simulink model "Test2_1"  (R2021a)
(part 1 of 2)
settings: Solver=FixedStepAuto  StartTime=0  StopTime=0.2  FixedStep=0.2  RelTol=1e-3
libraries: spsDistributedParametersLineLib x92, spsThreePhaseSeriesRLCLoadLib x30, spsThreePhaseVIMeasurementLib x4, spsGroundLib x1, spsThreePhaseSourceLib x1, spsSeriesRLCBranchLib x1, spspowerguiLib x1
settings Model: Creator=Admin  LastModifiedBy=Admin

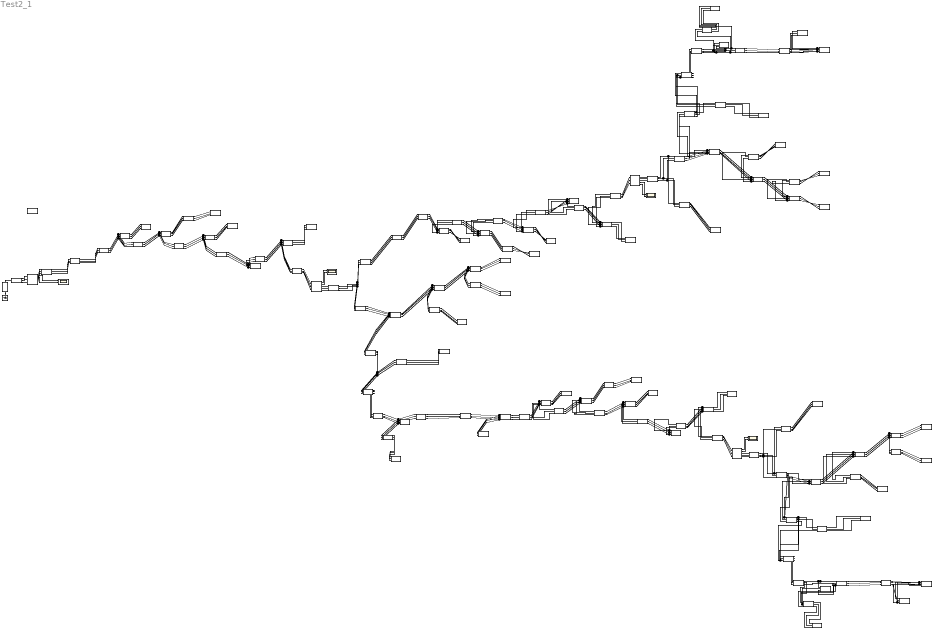
== system Test2_1 ==
  Ground : spsGroundLib/Ground  LConnTagsString=a
  Line 1 : spsDistributedParametersLineLib/Distributed Parameters Line  Phases=3  Length=1.11  Frequency=50  Resistance=[0.502970710632245 0.0486237908083191 0.0486712220507153;0.0486237908083191 0.502875844822084 0.0486237934466192;0.0486712220507153 0.0486237934466192 0.502970710632245]  Inductance=[0.00286900545038753 0.00133270803418135 0.00132951476746136;0.00133270803418135 0.00286931445999602 0.00133799988507366;0.00132951476746136 0.00133799988507366 0.00286900545038753]  Capacitance=[8.11484299003193e-09 -1.94249816214699e-09 -1.86930692621136e-09;-1.94249816214699e-09 8.0425699231653e-09 -1.98049571960044e-09;-1.86930692621136e-09 -1.98049571960044e-09 8.13337738722527e-09]  x1=[183.490948188185 4216.96054972605 4216.80340700784;314.159265358979 314.159265358979 314.159265358979;0.881345582847074 1.88304842426721 -2.82810315151267]  x2=[183.491209806206 4216.96449324722 4216.80735926271;314.159265358979 314.159265358979 314.159265358979;0.881345090635743 1.88304754646511 -2.82810403687592]  x3=[0.160865210922633 10.7270372245128 10.8089995229869;314.159265358979 314.159265358979 314.159265358979;0.879656680482595 1.88168039127429 -2.82947272736112]  x4=[0.160865210931406 10.7270372277551 10.8089995262806;314.159265358979 314.159265358979 314.159265358979;0.881345090559868 1.88304754646581 -2.82810403687496]  x5=5.37516004033389e-06  V1=ones(3,3)  V2=ones(3,3)  I1=ones(3,3)  I2=ones(3,3)  nHarmo=1  Measurements=None  Decoupling=off  VsMag0=0  VrMag0=0  VsAngle0=0  VrAngle0=0  IsMag0=0  IrMag0=0  IsAngle0=0  IrAngle0=0
      settings: SourceProductBaseCode=PS
  Line 10 : spsDistributedParametersLineLib/Distributed Parameters Line  Phases=3  Length=0.02  Frequency=50  Resistance=[0.646656091154803 0.0486237908083191 0.0486712220507153;0.0486237908083191 0.646561225344642 0.0486237934466192;0.0486712220507153 0.0486237934466192 0.646656091154803]  Inductance=[0.00282448912315926 0.00133270803418135 0.00132951476746136;0.00133270803418135 0.00282479813276775 0.00133799988507366;0.00132951476746136 0.00133799988507366 0.00282448912315926]  Capacitance=[7.89543174552926e-09 -1.85986777702161e-09 -1.7901190036642e-09;-1.85986777702161e-09 7.82540023894543e-09 -1.8957321828871e-09;-1.7901190036642e-09 -1.8957321828871e-09 7.91264394645417e-09]  x1=[139.613623241474 4217.53984964851 4217.63905801798;314.159265358979 314.159265358979 314.159265358979;0.931224583642913 1.89080283160816 -2.82029492609255]  x2=[139.613784628439 4217.52722308047 4217.62642474081;314.159265358979 314.159265358979 314.159265358979;0.931225166408948 1.89080004922946 -2.8202976922573]  x3=[0.125802639978614 9.6038595201039 9.68625501655352;314.159265358979 314.159265358979 314.159265358979;0.906622980836671 1.88104314108493 -2.82997412629294]  x4=[0.118411687429991 11.8627957177303 11.9457690734741;314.159265358979 314.159265358979 314.159265358979;0.957331649560871 1.89867986271673 -2.81247074601716]  x5=9.5829454252223e-08  V1=ones(3,3)  V2=ones(3,3)  I1=ones(3,3)  I2=ones(3,3)  nHarmo=1  Measurements=None  Decoupling=off  VsMag0=0  VrMag0=0  VsAngle0=0  VrAngle0=0  IsMag0=0  IrMag0=0  IsAngle0=0  IrAngle0=0
      settings: SourceProductBaseCode=PS
  Line 11 : spsDistributedParametersLineLib/Distributed Parameters Line  Phases=3  Length=1.15  Frequency=50  Resistance=[0.646656091154803 0.0486237908083191 0.0486712220507153;0.0486237908083191 0.646561225344642 0.0486237934466192;0.0486712220507153 0.0486237934466192 0.646656091154803]  Inductance=[0.00282448912315926 0.00133270803418135 0.00132951476746136;0.00133270803418135 0.00282479813276775 0.00133799988507366;0.00132951476746136 0.00133799988507366 0.00282448912315926]  Capacitance=[7.89543174552926e-09 -1.85986777702161e-09 -1.7901190036642e-09;-1.85986777702161e-09 7.82540023894543e-09 -1.8957321828871e-09;-1.7901190036642e-09 -1.8957321828871e-09 7.91264394645417e-09]  x1=[139.613623241474 4217.53984964851 4217.63905801798;314.159265358979 314.159265358979 314.159265358979;0.929523610974372 1.8894515205395 -2.82164752351366]  x2=[139.617533988018 4216.93608513133 4217.03622024235;314.159265358979 314.159265358979 314.159265358979;0.929545542963053 1.88940575482222 -2.82169270993868]  x3=[0.124028196256623 10.0434970519779 10.1259039409958;314.159265358979 314.159265358979 314.159265358979;0.91978125610013 1.91390155222964 -2.79739650737982]  x4=[0.119986768860265 11.3991555600104 11.4816493598603;314.159265358979 314.159265358979 314.159265358979;0.937855860263933 1.86657270231703 -2.84437284120632]  x5=5.51019361950282e-06  V1=ones(3,3)  V2=ones(3,3)  I1=ones(3,3)  I2=ones(3,3)  nHarmo=1  Measurements=None  Decoupling=off  VsMag0=0  VrMag0=0  VsAngle0=0  VrAngle0=0  IsMag0=0  IrMag0=0  IsAngle0=0  IrAngle0=0
      settings: SourceProductBaseCode=PS
  Line 12 : spsDistributedParametersLineLib/Distributed Parameters Line  Phases=3  Length=0.18999  Frequency=50  Resistance=[0.646656091154803 0.0486237908083191 0.0486712220507153;0.0486237908083191 0.646561225344642 0.0486237934466192;0.0486712220507153 0.0486237934466192 0.646656091154803]  Inductance=[0.00282448912315926 0.00133270803418135 0.00132951476746136;0.00133270803418135 0.00282479813276775 0.00133799988507366;0.00132951476746136 0.00133799988507366 0.00282448912315926]  Capacitance=[7.89543174552926e-09 -1.85986777702161e-09 -1.7901190036642e-09;-1.85986777702161e-09 7.82540023894543e-09 -1.8957321828871e-09;-1.7901190036642e-09 -1.8957321828871e-09 7.91264394645417e-09]  x1=[139.617533988018 4216.93608513133 4217.03622024235;314.159265358979 314.159265358979 314.159265358979;0.930990632141395 1.89055378326383 -2.82054358865528]  x2=[139.617810696745 4216.88803294502 4216.98826109063;314.159265358979 314.159265358979 314.159265358979;0.930992215475269 1.89055205647319 -2.82054527154911]  x3=[0.122939571492091 10.4380099860844 10.5206430059255;314.159265358979 314.159265358979 314.159265358979;0.927045766208167 1.90632955416081 -2.80488079283943]  x4=[0.121184863909517 11.0230596059142 11.1057028683583;314.159265358979 314.159265358979 314.159265358979;0.934706144543507 1.87539251063379 -2.83560426898356]  x5=9.10331900668992e-07  V1=ones(3,3)  V2=ones(3,3)  I1=ones(3,3)  I2=ones(3,3)  nHarmo=1  Measurements=None  Decoupling=off  VsMag0=0  VrMag0=0  VsAngle0=0  VrAngle0=0  IsMag0=0  IrMag0=0  IsAngle0=0  IrAngle0=0
      settings: SourceProductBaseCode=PS
  Line 13 : spsDistributedParametersLineLib/Distributed Parameters Line  Phases=3  Length=0.34003  Frequency=50  Resistance=[0.646656091154803 0.0486237908083191 0.0486712220507153;0.0486237908083191 0.646561225344642 0.0486237934466192;0.0486712220507153 0.0486237934466192 0.646656091154803]  Inductance=[0.00282448912315926 0.00133270803418135 0.00132951476746136;0.00133270803418135 0.00282479813276775 0.00133799988507366;0.00132951476746136 0.00133799988507366 0.00282448912315926]  Capacitance=[7.89543174552926e-09 -1.85986777702161e-09 -1.7901190036642e-09;-1.85986777702161e-09 7.82540023894543e-09 -1.8957321828871e-09;-1.7901190036642e-09 -1.8957321828871e-09 7.91264394645417e-09]  x1=[139.617533988018 4216.93608513133 4217.03622024235;314.159265358979 314.159265358979 314.159265358979;0.930764779097866 1.89037435785433 -2.82072318486507]  x2=[139.618104729463 4216.84184429517 4216.94208355787;314.159265358979 314.159265358979 314.159265358979;0.93076870908045 1.89036443392397 -2.82073301164643]  x3=[0.123198048363616 10.3414524616606 10.4240238869745;314.159265358979 314.159265358979 314.159265358979;0.926605418652431 1.89963559608898 -2.81153392755128]  x4=[0.12090892368481 11.1141558874419 11.1968133364116;314.159265358979 314.159265358979 314.159265358979;0.93449013875314 1.88135489849309 -2.82968069963196]  x5=1.62924446646917e-06  V1=ones(3,3)  V2=ones(3,3)  I1=ones(3,3)  I2=ones(3,3)  nHarmo=1  Measurements=None  Decoupling=off  VsMag0=0  VrMag0=0  VsAngle0=0  VrAngle0=0  IsMag0=0  IrMag0=0  IsAngle0=0  IrAngle0=0
      settings: SourceProductBaseCode=PS
  Line 14 : spsDistributedParametersLineLib/Distributed Parameters Line  Phases=3  Length=0.12001  Frequency=50  Resistance=[0.646656091154803 0.0486237908083191 0.0486712220507153;0.0486237908083191 0.646561225344642 0.0486237934466192;0.0486712220507153 0.0486237934466192 0.646656091154803]  Inductance=[0.00282448912315926 0.00133270803418135 0.00132951476746136;0.00133270803418135 0.00282479813276775 0.00133799988507366;0.00132951476746136 0.00133799988507366 0.00282448912315926]  Capacitance=[7.89543174552926e-09 -1.85986777702161e-09 -1.7901190036642e-09;-1.85986777702161e-09 7.82540023894543e-09 -1.8957321828871e-09;-1.7901190036642e-09 -1.8957321828871e-09 7.91264394645417e-09]  x1=[139.618104729463 4216.84184429517 4216.94208355787;314.159265358979 314.159265358979 314.159265358979;0.931099902006585 1.8906275449517 -2.82046965015564]  x2=[139.618198251544 4216.82534126711 4216.9256107533;314.159265358979 314.159265358979 314.159265358979;0.931100467134369 1.89062683124206 -2.82047034850588]  x3=[0.122552692495042 10.5677297439231 10.6503804943866;314.159265358979 314.159265358979 314.159265358979;0.929028818858428 1.89867493848402 -2.81247897616698]  x4=[0.121579589071698 10.8927747635657 10.9754353650445;314.159265358979 314.159265358979 314.159265358979;0.933006753373057 1.88267821187084 -2.82836588068453]  x5=5.75024640240464e-07  V1=ones(3,3)  V2=ones(3,3)  I1=ones(3,3)  I2=ones(3,3)  nHarmo=1  Measurements=None  Decoupling=off  VsMag0=0  VrMag0=0  VsAngle0=0  VrAngle0=0  IsMag0=0  IrMag0=0  IsAngle0=0  IrAngle0=0
      settings: SourceProductBaseCode=PS
  Line 15 : spsDistributedParametersLineLib/Distributed Parameters Line  Phases=3  Length=0.82  Frequency=50  Resistance=[0.646656091154803 0.0486237908083191 0.0486712220507153;0.0486237908083191 0.646561225344642 0.0486237934466192;0.0486712220507153 0.0486237934466192 0.646656091154803]  Inductance=[0.00282448912315926 0.00133270803418135 0.00132951476746136;0.00133270803418135 0.00282479813276775 0.00133799988507366;0.00132951476746136 0.00133799988507366 0.00282448912315926]  Capacitance=[7.89543174552926e-09 -1.85986777702161e-09 -1.7901190036642e-09;-1.85986777702161e-09 7.82540023894543e-09 -1.8957321828871e-09;-1.7901190036642e-09 -1.8957321828871e-09 7.91264394645417e-09]  x1=[139.618104729463 4216.84184429517 4216.94208355787;314.159265358979 314.159265358979 314.159265358979;0.930046217176273 1.88979046155794 -2.82130753039351]  x2=[139.618676062845 4216.72417533179 4216.8244531276;314.159265358979 314.159265358979 314.159265358979;0.930052345912838 1.88977235992586 -2.82132549460337]  x3=[0.12268247979231 10.4975028788883 10.5799917950037;314.159265358979 314.159265358979 314.159265358979;0.928447585932489 1.89122880253881 -2.81988123007282]  x4=[0.121366717303898 10.9449655935799 11.0275286658794;314.159265358979 314.159265358979 314.159265358979;0.930427151352339 1.88743234081576 -2.82365546167697]  x5=3.92900762434114e-06  V1=ones(3,3)  V2=ones(3,3)  I1=ones(3,3)  I2=ones(3,3)  nHarmo=1  Measurements=None  Decoupling=off  VsMag0=0  VrMag0=0  VsAngle0=0  VrAngle0=0  IsMag0=0  IrMag0=0  IsAngle0=0  IrAngle0=0
      settings: SourceProductBaseCode=PS
  Line 16 : spsDistributedParametersLineLib/Distributed Parameters Line  Phases=3  Length=1.11  Frequency=50  Resistance=[0.646656091154803 0.0486237908083191 0.0486712220507153;0.0486237908083191 0.646561225344642 0.0486237934466192;0.0486712220507153 0.0486237934466192 0.646656091154803]  Inductance=[0.00282448912315926 0.00133270803418135 0.00132951476746136;0.00133270803418135 0.00282479813276775 0.00133799988507366;0.00132951476746136 0.00133799988507366 0.00282448912315926]  Capacitance=[7.89543174552926e-09 -1.85986777702161e-09 -1.7901190036642e-09;-1.85986777702161e-09 7.82540023894543e-09 -1.8957321828871e-09;-1.7901190036642e-09 -1.8957321828871e-09 7.91264394645417e-09]  x1=[139.600491467484 4218.81584590393 4218.91451607418;314.159265358979 314.159265358979 314.159265358979;0.929531540696171 1.88970018528801 -2.82140025221224]  x2=[139.613623241474 4217.53984964851 4217.63905801798;314.159265358979 314.159265358979 314.159265358979;0.929583822396267 1.88949935455963 -2.82159964395893]  x3=[0.127788296873858 8.91671166939087 8.99888036016685;314.159265358979 314.159265358979 314.159265358979;0.894267153933206 1.90517971225722 -2.80607870861062]  x4=[0.116365696912827 12.5277305076564 12.6105347462274;314.159265358979 314.159265358979 314.159265358979;0.966560726223664 1.87737433079823 -2.83364315743487]  x5=5.31853471099837e-06  V1=ones(3,3)  V2=ones(3,3)  I1=ones(3,3)  I2=ones(3,3)  nHarmo=1  Measurements=None  Decoupling=off  VsMag0=0  VrMag0=0  VsAngle0=0  VrAngle0=0  IsMag0=0  IrMag0=0  IsAngle0=0  IrAngle0=0
      settings: SourceProductBaseCode=PS
  Line 17 : spsDistributedParametersLineLib/Distributed Parameters Line  Phases=3  Length=0.20999  Frequency=50  Resistance=[0.646656091154803 0.0486237908083191 0.0486712220507153;0.0486237908083191 0.646561225344642 0.0486237934466192;0.0486712220507153 0.0486237934466192 0.646656091154803]  Inductance=[0.00282448912315926 0.00133270803418135 0.00132951476746136;0.00133270803418135 0.00282479813276775 0.00133799988507366;0.00132951476746136 0.00133799988507366 0.00282448912315926]  Capacitance=[7.89543174552926e-09 -1.85986777702161e-09 -1.7901190036642e-09;-1.85986777702161e-09 7.82540023894543e-09 -1.8957321828871e-09;-1.7901190036642e-09 -1.8957321828871e-09 7.91264394645417e-09]  x1=[139.600491467484 4218.81584590393 4218.91451607418;314.159265358979 314.159265358979 314.159265358979;0.93088631274167 1.89077646269943 -2.82032295026095]  x2=[139.60098568848 4218.8374405526 4218.93595905468;314.159265358979 314.159265358979 314.159265358979;0.930885554137233 1.89076995286526 -2.82032946246903]  x3=[0.122301871680709 10.7361501200076 10.81871266322;314.159265358979 314.159265358979 314.159265358979;0.920433370592123 1.87027382272559 -2.84067456788957]  x4=[0.121801775748973 10.7360630313458 10.8188196037761;314.159265358979 314.159265358979 314.159265358979;0.941064659483104 1.91102162140943 -2.80022942069814]  x5=1.00616135492121e-06  V1=ones(3,3)  V2=ones(3,3)  I1=ones(3,3)  I2=ones(3,3)  nHarmo=1  Measurements=None  Decoupling=off  VsMag0=0  VrMag0=0  VsAngle0=0  VrAngle0=0  IsMag0=0  IrMag0=0  IsAngle0=0  IrAngle0=0
      settings: SourceProductBaseCode=PS
  Line 18 : spsDistributedParametersLineLib/Distributed Parameters Line  Phases=3  Length=0.23001  Frequency=50  Resistance=[0.476003738225748 0.351747138225748 0.351747138225748;0.351747138225748 0.476003738225748 0.351747138225748;0.351747138225748 0.351747138225748 0.476003738225748]  Inductance=[0.000705954362986426 0.000459934243504405 0.000459934243504405;0.000459934243504405 0.000705954362986426 0.000459934243504405;0.000459934243504405 0.000459934243504405 0.000705954362986426]  Capacitance=[5.7561313269996e-07 -1.37543883484145e-07 -1.37543912800485e-07;-1.37543883484145e-07 5.75613027339387e-07 -1.37543875208088e-07;-1.37543912800485e-07 -1.37543875208088e-07 5.75613005057695e-07]  x1=[87.2243517312692 4219.54153891526 4219.23920669129;314.159265358979 314.159265358979 314.159265358979;1.07727319320854 1.8084440090155 -2.90287048996644]  x2=[87.2244629956902 4219.54347170392 4219.24113933993;314.159265358979 314.159265358979 314.159265358979;1.07727024748328 1.80844327260835 -2.90287122637374]  x3=[1.18260840704652 226.919360409331 226.90308395695;314.159265358979 314.159265358979 314.159265358979;1.07567446634063 1.80748650298844 -2.9038279959571]  x4=[1.18260840611565 226.919360397577 226.903084041185;314.159265358979 314.159265358979 314.159265358979;1.07727024853953 1.80844327260969 -2.90287122633514]  x5=5.08421409621804e-06  V1=ones(3,3)  V2=ones(3,3)  I1=ones(3,3)  I2=ones(3,3)  nHarmo=1  Measurements=None  Decoupling=off  VsMag0=0  VrMag0=0  VsAngle0=0  VrAngle0=0  IsMag0=0  IrMag0=0  IsAngle0=0  IrAngle0=0
      settings: SourceProductBaseCode=PS
  Line 19 : spsDistributedParametersLineLib/Distributed Parameters Line  Phases=3  Length=0.24001  Frequency=50  Resistance=[0.646656091154803 0.0486237908083191 0.0486712220507153;0.0486237908083191 0.646561225344642 0.0486237934466192;0.0486712220507153 0.0486237934466192 0.646656091154803]  Inductance=[0.00282448912315926 0.00133270803418135 0.00132951476746136;0.00133270803418135 0.00282479813276775 0.00133799988507366;0.00132951476746136 0.00133799988507366 0.00282448912315926]  Capacitance=[7.89543174552926e-09 -1.85986777702161e-09 -1.7901190036642e-09;-1.85986777702161e-09 7.82540023894543e-09 -1.8957321828871e-09;-1.7901190036642e-09 -1.8957321828871e-09 7.91264394645417e-09]  x1=[139.601103101959 4219.06510568206 4219.16605914604;314.159265358979 314.159265358979 314.159265358979;0.93081961734594 1.89079206583915 -2.82030799120796]  x2=[139.600491467614 4218.81584590389 4218.91451607394;314.159265358979 314.159265358979 314.159265358979;0.930841124072783 1.89074056326736 -2.82035888386677]  x3=[0.127690286518134 8.92547553801441 9.00231366385189;314.159265358979 314.159265358979 314.159265358979;0.961115303635879 1.88030971985997 -2.82927506920421]  x4=[0.116521098887311 12.5429375526517 12.6312344689864;314.159265358979 314.159265358979 314.159265358979;0.89726280865193 1.89796144882471 -2.81420679508576]  x5=1.1500013657538e-06  V1=ones(3,3)  V2=ones(3,3)  I1=ones(3,3)  I2=ones(3,3)  nHarmo=1  Measurements=None  Decoupling=off  VsMag0=0  VrMag0=0  VsAngle0=0  VrAngle0=0  IsMag0=0  IrMag0=0  IsAngle0=0  IrAngle0=0
      settings: SourceProductBaseCode=PS
  Line 2 : spsDistributedParametersLineLib/Distributed Parameters Line  Phases=3  Length=0.03  Frequency=50  Resistance=[0.476003738225748 0.351747138225748 0.351747138225748;0.351747138225748 0.476003738225748 0.351747138225748;0.351747138225748 0.351747138225748 0.476003738225748]  Inductance=[0.000705954362986426 0.000459934243504405 0.000459934243504405;0.000459934243504405 0.000705954362986426 0.000459934243504405;0.000459934243504405 0.000459934243504405 0.000705954362986426]  Capacitance=[5.7561313269996e-07 -1.37543883484145e-07 -1.37543912800485e-07;-1.37543883484145e-07 5.75613027339387e-07 -1.37543875208088e-07;-1.37543912800485e-07 -1.37543875208088e-07 5.75613005057695e-07]  x1=[87.2784474669042 4217.75377370592 4217.44930563501;314.159265358979 314.159265358979 314.159265358979;1.0788854371739 1.80887693912269 -2.90243540997328]  x2=[87.2784519303965 4217.75384057205 4217.44937290109;314.159265358979 314.159265358979 314.159265358979;1.07888527907257 1.80887691360674 -2.90243543558482]  x3=[1.18615398682892 227.050829720101 227.034451809516;314.159265358979 314.159265358979 314.159265358979;1.07846570612573 1.80868741549984 -2.90262549147584]  x4=[1.18622591389486 227.050858783612 227.034421297238;314.159265358979 314.159265358979 314.159265358979;1.07909663787919 1.8089415923141 -2.9023701989552]  x5=6.63129528657629e-07  V1=ones(3,3)  V2=ones(3,3)  I1=ones(3,3)  I2=ones(3,3)  nHarmo=1  Measurements=None  Decoupling=off  VsMag0=0  VrMag0=0  VsAngle0=0  VrAngle0=0  IsMag0=0  IrMag0=0  IsAngle0=0  IrAngle0=0
      settings: SourceProductBaseCode=PS
  Line 20 : spsDistributedParametersLineLib/Distributed Parameters Line  Phases=3  Length=0.02  Frequency=50  Resistance=[0.646656091154803 0.0486237908083191 0.0486712220507153;0.0486237908083191 0.646561225344642 0.0486237934466192;0.0486712220507153 0.0486237934466192 0.646656091154803]  Inductance=[0.00282448912315926 0.00133270803418135 0.00132951476746136;0.00133270803418135 0.00282479813276775 0.00133799988507366;0.00132951476746136 0.00133799988507366 0.00282448912315926]  Capacitance=[7.89543174552926e-09 -1.85986777702161e-09 -1.7901190036642e-09;-1.85986777702161e-09 7.82540023894543e-09 -1.8957321828871e-09;-1.7901190036642e-09 -1.8957321828871e-09 7.91264394645417e-09]  x1=[139.601103101959 4219.06510568207 4219.16605914604;314.159265358979 314.159265358979 314.159265358979;0.931150795219219 1.89105516490837 -2.82004464168706]  x2=[139.601114137607 4219.06259404817 4219.1635493867;314.159265358979 314.159265358979 314.159265358979;0.931150916152489 1.89105487509985 -2.82004492869826]  x3=[0.122586926612653 10.5573636449377 10.6400601112212;314.159265358979 314.159265358979 314.159265358979;0.930385694308767 1.89472208249132 -2.81639985048892]  x4=[0.121527025725859 10.9163955079092 10.9991421429457;314.159265358979 314.159265358979 314.159265358979;0.931892453418219 1.88748504102292 -2.82359427469835]  x5=9.5829454252223e-08  V1=ones(3,3)  V2=ones(3,3)  I1=ones(3,3)  I2=ones(3,3)  nHarmo=1  Measurements=None  Decoupling=off  VsMag0=0  VrMag0=0  VsAngle0=0  VrAngle0=0  IsMag0=0  IrMag0=0  IsAngle0=0  IrAngle0=0
      settings: SourceProductBaseCode=PS
  Line 21 : spsDistributedParametersLineLib/Distributed Parameters Line  Phases=3  Length=0.5  Frequency=50  Resistance=[0.646656091154803 0.0486237908083191 0.0486712220507153;0.0486237908083191 0.646561225344642 0.0486237934466192;0.0486712220507153 0.0486237934466192 0.646656091154803]  Inductance=[0.00282448912315926 0.00133270803418135 0.00132951476746136;0.00133270803418135 0.00282479813276775 0.00133799988507366;0.00132951476746136 0.00133799988507366 0.00282448912315926]  Capacitance=[7.89543174552926e-09 -1.85986777702161e-09 -1.7901190036642e-09;-1.85986777702161e-09 7.82540023894543e-09 -1.8957321828871e-09;-1.7901190036642e-09 -1.8957321828871e-09 7.91264394645417e-09]  x1=[139.602041514112 4219.64605914901 4219.75171929061;314.159265358979 314.159265358979 314.159265358979;0.930380617159176 1.89059601798522 -2.82050567255881]  x2=[139.601103101959 4219.06510568206 4219.16605914604;314.159265358979 314.159265358979 314.159265358979;0.930428258156476 1.89048115666682 -2.82061919634381]  x3=[0.128199187090919 8.74438863690465 8.82122942129422;314.159265358979 314.159265358979 314.159265358979;0.959107105240511 1.88361656679194 -2.82596842987331]  x4=[0.115972595804543 12.7192802215745 12.8075977373578;314.159265358979 314.159265358979 314.159265358979;0.897882359224302 1.89479280951018 -2.81734450846133]  x5=2.39573635630557e-06  V1=ones(3,3)  V2=ones(3,3)  I1=ones(3,3)  I2=ones(3,3)  nHarmo=1  Measurements=None  Decoupling=off  VsMag0=0  VrMag0=0  VsAngle0=0  VrAngle0=0  IsMag0=0  IrMag0=0  IsAngle0=0  IrAngle0=0
      settings: SourceProductBaseCode=PS
  Line 22 : spsDistributedParametersLineLib/Distributed Parameters Line  Phases=3  Length=0.23  Frequency=50  Resistance=[0.646656091154803 0.0486237908083191 0.0486712220507153;0.0486237908083191 0.646561225344642 0.0486237934466192;0.0486712220507153 0.0486237934466192 0.646656091154803]  Inductance=[0.00282448912315926 0.00133270803418135 0.00132951476746136;0.00133270803418135 0.00282479813276775 0.00133799988507366;0.00132951476746136 0.00133799988507366 0.00282448912315926]  Capacitance=[7.89543174552926e-09 -1.85986777702161e-09 -1.7901190036642e-09;-1.85986777702161e-09 7.82540023894543e-09 -1.8957321828871e-09;-1.7901190036642e-09 -1.8957321828871e-09 7.91264394645417e-09]  x1=[139.601723058153 4220.08455899527 4220.192279394;314.159265358979 314.159265358979 314.159265358979;0.930756622759197 1.89099330692861 -2.82010888561997]  x2=[139.602041514112 4219.64605914901 4219.75171929061;314.159265358979 314.159265358979 314.159265358979;0.930787044256969 1.89091889762109 -2.82018248556439]  x3=[0.131418967401202 7.65799205551827 7.73504268799798;314.159265358979 314.159265358979 314.159265358979;0.955113070612998 1.90880560013735 -2.80076263531449]  x4=[0.112756825248139 13.8164851234199 13.9052284500049;314.159265358979 314.159265358979 314.159265358979;0.902026023744351 1.88084936289819 -2.83114163465159]  x5=1.10203872390056e-06  V1=ones(3,3)  V2=ones(3,3)  I1=ones(3,3)  I2=ones(3,3)  nHarmo=1  Measurements=None  Decoupling=off  VsMag0=0  VrMag0=0  VsAngle0=0  VrAngle0=0  IsMag0=0  IrMag0=0  IsAngle0=0  IrAngle0=0
      settings: SourceProductBaseCode=PS
  Line 23 : spsDistributedParametersLineLib/Distributed Parameters Line  Phases=3  Length=1.62  Frequency=50  Resistance=[0.80718830189013 0.0486237908083191 0.0486712220507153;0.0486237908083191 0.807093436079969 0.0486237934466192;0.0486712220507153 0.0486237934466192 0.80718830189013]  Inductance=[0.00279786707424938 0.00133270803418135 0.00132951476746136;0.00133270803418135 0.00279817608385787 0.00133799988507366;0.00132951476746136 0.00133799988507366 0.00279786707424938]  Capacitance=[7.73340098830622e-09 -1.79942827973291e-09 -1.73218055098733e-09;-1.79942827973291e-09 7.66505189233746e-09 -1.83375898618858e-09;-1.73218055098733e-09 -1.83375898618858e-09 7.749673531177e-09]  x1=[107.448176831119 4220.17320978757 4220.46007124655;314.159265358979 314.159265358979 314.159265358979;0.988833228344866 1.89366453122739 -2.81742079155062]  x2=[107.448651192593 4220.1679328506 4220.45483223968;314.159265358979 314.159265358979 314.159265358979;0.988832200124081 1.89366176084507 -2.81742357698124]  x3=[0.0935875110467654 10.6803147710633 10.762324591659;314.159265358979 314.159265358979 314.159265358979;0.986020401016198 1.89224326860657 -2.8188469892252]  x4=[0.0935090241097448 10.6949899335453 10.7769992356585;314.159265358979 314.159265358979 314.159265358979;0.98922518520354 1.89318284867866 -2.81789917072241]  x5=7.70442045759223e-06  V1=ones(3,3)  V2=ones(3,3)  I1=ones(3,3)  I2=ones(3,3)  nHarmo=1  Measurements=None  Decoupling=off  VsMag0=0  VrMag0=0  VsAngle0=0  VrAngle0=0  IsMag0=0  IrMag0=0  IsAngle0=0  IrAngle0=0
      settings: SourceProductBaseCode=PS
  Line 24 : spsDistributedParametersLineLib/Distributed Parameters Line  Phases=3  Length=0.54002  Frequency=50  Resistance=[0.646656091154803 0.0486237908083191 0.0486712220507153;0.0486237908083191 0.646561225344642 0.0486237934466192;0.0486712220507153 0.0486237934466192 0.646656091154803]  Inductance=[0.00282448912315926 0.00133270803418135 0.00132951476746136;0.00133270803418135 0.00282479813276775 0.00133799988507366;0.00132951476746136 0.00133799988507366 0.00282448912315926]  Capacitance=[7.89543174552926e-09 -1.85986777702161e-09 -1.7901190036642e-09;-1.85986777702161e-09 7.82540023894543e-09 -1.8957321828871e-09;-1.7901190036642e-09 -1.8957321828871e-09 7.91264394645417e-09]  x1=[139.600619384139 4221.11147533114 4221.22401178701;314.159265358979 314.159265358979 314.159265358979;0.93021944834039 1.8907991987903 -2.82030523367007]  x2=[139.601723058153 4220.08455899527 4220.192279394;314.159265358979 314.159265358979 314.159265358979;0.930289954133797 1.8906225693556 -2.8204799761089]  x3=[0.131411960666678 7.64984266223699 7.72683853675604;314.159265358979 314.159265358979 314.159265358979;0.951519598066089 1.90580424954729 -2.80376720147912]  x4=[0.11270709337898 13.8202545776016 13.9089289920831;314.159265358979 314.159265358979 314.159265358979;0.904579557057469 1.88185487223023 -2.8301310503581]  x5=2.58749109426427e-06  V1=ones(3,3)  V2=ones(3,3)  I1=ones(3,3)  I2=ones(3,3)  nHarmo=1  Measurements=None  Decoupling=off  VsMag0=0  VrMag0=0  VsAngle0=0  VrAngle0=0  IsMag0=0  IrMag0=0  IsAngle0=0  IrAngle0=0
      settings: SourceProductBaseCode=PS
  Line 25 : spsDistributedParametersLineLib/Distributed Parameters Line  Phases=3  Length=0.13998  Frequency=50  Resistance=[0.646656091154803 0.0486237908083191 0.0486712220507153;0.0486237908083191 0.646561225344642 0.0486237934466192;0.0486712220507153 0.0486237934466192 0.646656091154803]  Inductance=[0.00282448912315926 0.00133270803418135 0.00132951476746136;0.00133270803418135 0.00282479813276775 0.00133799988507366;0.00132951476746136 0.00133799988507366 0.00282448912315926]  Capacitance=[7.89543174552926e-09 -1.85986777702161e-09 -1.7901190036642e-09;-1.85986777702161e-09 7.82540023894543e-09 -1.8957321828871e-09;-1.7901190036642e-09 -1.8957321828871e-09 7.91264394645417e-09]  x1=[139.600619384139 4221.11147533114 4221.22401178701;314.159265358979 314.159265358979 314.159265358979;0.930821622770765 1.89127758682561 -2.81982639024322]  x2=[139.601368793916 4221.03275764691 4221.14543470752;314.159265358979 314.159265358979 314.159265358979;0.930823757939632 1.89127416145099 -2.81982974209551]  x3=[0.12424213815074 10.0813098041737 10.1640019037911;314.159265358979 314.159265358979 314.159265358979;0.913233828554971 1.92592809161701 -2.78542877628517]  x4=[0.119895951623731 11.4110428279263 11.4938192732766;314.159265358979 314.159265358979 314.159265358979;0.94883467665136 1.86050539709626 -2.85040396273424]  x5=6.70710350311308e-07  V1=ones(3,3)  V2=ones(3,3)  I1=ones(3,3)  I2=ones(3,3)  nHarmo=1  Measurements=None  Decoupling=off  VsMag0=0  VrMag0=0  VsAngle0=0  VrAngle0=0  IsMag0=0  IrMag0=0  IsAngle0=0  IrAngle0=0
      settings: SourceProductBaseCode=PS
  Line 26 : spsDistributedParametersLineLib/Distributed Parameters Line  Phases=3  Length=0.14996  Frequency=50  Resistance=[0.476003738225748 0.351747138225748 0.351747138225748;0.351747138225748 0.476003738225748 0.351747138225748;0.351747138225748 0.351747138225748 0.476003738225748]  Inductance=[0.000705954362986426 0.000459934243504405 0.000459934243504405;0.000459934243504405 0.000705954362986426 0.000459934243504405;0.000459934243504405 0.000459934243504405 0.000705954362986426]  Capacitance=[5.7561313269996e-07 -1.37543883484145e-07 -1.37543912800485e-07;-1.37543883484145e-07 5.75613027339387e-07 -1.37543875208088e-07;-1.37543912800485e-07 -1.37543875208088e-07 5.75613005057695e-07]  x1=[87.186146373575 4221.73596477474 4221.45032772977;314.159265358979 314.159265358979 314.159265358979;1.07744325027428 1.80919730311081 -2.90212110156354]  x2=[87.1861936446919 4221.71867570315 4221.43303982852;314.159265358979 314.159265358979 314.159265358979;1.07744199810758 1.80919733969441 -2.90212106497979]  x3=[1.18322786523239 226.463783195717 226.448443450913;314.159265358979 314.159265358979 314.159265358979;1.07640125231192 1.81074727542554 -2.90057112903511]  x4=[1.18322790616703 227.793026104387 227.777596349487;314.159265358979 314.159265358979 314.159265358979;1.0774420063186 1.80703404976602 -2.90428435507242]  x5=3.31476347058327e-06  V1=ones(3,3)  V2=ones(3,3)  I1=ones(3,3)  I2=ones(3,3)  nHarmo=1  Measurements=None  Decoupling=off  VsMag0=0  VrMag0=0  VsAngle0=0  VrAngle0=0  IsMag0=0  IrMag0=0  IsAngle0=0  IrAngle0=0
      settings: SourceProductBaseCode=PS
  Line 27 : spsDistributedParametersLineLib/Distributed Parameters Line  Phases=3  Length=0.50001  Frequency=50  Resistance=[0.646656091154803 0.0486237908083191 0.0486712220507153;0.0486237908083191 0.646561225344642 0.0486237934466192;0.0486712220507153 0.0486237934466192 0.646656091154803]  Inductance=[0.00282448912315926 0.00133270803418135 0.00132951476746136;0.00133270803418135 0.00282479813276775 0.00133799988507366;0.00132951476746136 0.00133799988507366 0.00282448912315926]  Capacitance=[7.89543174552926e-09 -1.85986777702161e-09 -1.7901190036642e-09;-1.85986777702161e-09 7.82540023894543e-09 -1.8957321828871e-09;-1.7901190036642e-09 -1.8957321828871e-09 7.91264394645417e-09]  x1=[139.596827955923 4222.34183377535 4222.45832100252;314.159265358979 314.159265358979 314.159265358979;0.930207051674438 1.8910232686144 -2.82008312290127]  x2=[139.600619384139 4221.11147533114 4221.22401178701;314.159265358979 314.159265358979 314.159265358979;0.930279674815143 1.89084704476893 -2.82025734214545]  x3=[0.133555604144539 7.00248497588752 7.07999691108018;314.159265358979 314.159265358979 314.159265358979;0.934123994453282 1.95650137074991 -2.75344987405581]  x4=[0.110499757176719 14.4954338851781 14.5844508131919;314.159265358979 314.159265358979 314.159265358979;0.924721783156691 1.85883547174202 -2.85298548818485]  x5=2.3957842710327e-06  V1=ones(3,3)  V2=ones(3,3)  I1=ones(3,3)  I2=ones(3,3)  nHarmo=1  Measurements=None  Decoupling=off  VsMag0=0  VrMag0=0  VsAngle0=0  VrAngle0=0  IsMag0=0  IrMag0=0  IsAngle0=0  IrAngle0=0
      settings: SourceProductBaseCode=PS
  Line 28 : spsDistributedParametersLineLib/Distributed Parameters Line  Phases=3  Length=0.17  Frequency=50  Resistance=[0.646656091154803 0.0486237908083191 0.0486712220507153;0.0486237908083191 0.646561225344642 0.0486237934466192;0.0486712220507153 0.0486237934466192 0.646656091154803]  Inductance=[0.00282448912315926 0.00133270803418135 0.00132951476746136;0.00133270803418135 0.00282479813276775 0.00133799988507366;0.00132951476746136 0.00133799988507366 0.00282448912315926]  Capacitance=[7.89543174552926e-09 -1.85986777702161e-09 -1.7901190036642e-09;-1.85986777702161e-09 7.82540023894543e-09 -1.8957321828871e-09;-1.7901190036642e-09 -1.8957321828871e-09 7.91264394645417e-09]  x1=[139.596827955923 4222.34183377535 4222.45832100252;314.159265358979 314.159265358979 314.159265358979;0.930703810957929 1.89141791123897 -2.81968810460486]  x2=[139.59749465379 4222.22364011042 4222.3403524044;314.159265358979 314.159265358979 314.159265358979;0.930707767968534 1.89141355225234 -2.81969235502765]  x3=[0.124470133612505 9.94686905369949 10.0295788089809;314.159265358979 314.159265358979 314.159265358979;0.920661325570911 1.936865182314 -2.77458025454019]  x4=[0.119631510017528 11.5586499729936 11.6414162790545;314.159265358979 314.159265358979 314.159265358979;0.940895445587795 1.8521183070642 -2.85874039678463]  x5=8.14550361143895e-07  V1=ones(3,3)  V2=ones(3,3)  I1=ones(3,3)  I2=ones(3,3)  nHarmo=1  Measurements=None  Decoupling=off  VsMag0=0  VrMag0=0  VsAngle0=0  VrAngle0=0  IsMag0=0  IrMag0=0  IsAngle0=0  IrAngle0=0
      settings: SourceProductBaseCode=PS
  Line 29 : spsDistributedParametersLineLib/Distributed Parameters Line  Phases=3  Length=0.27998  Frequency=50  Resistance=[0.646656091154803 0.0486237908083191 0.0486712220507153;0.0486237908083191 0.646561225344642 0.0486237934466192;0.0486712220507153 0.0486237934466192 0.646656091154803]  Inductance=[0.00282448912315926 0.00133270803418135 0.00132951476746136;0.00133270803418135 0.00282479813276775 0.00133799988507366;0.00132951476746136 0.00133799988507366 0.00282448912315926]  Capacitance=[7.89543174552926e-09 -1.85986777702161e-09 -1.7901190036642e-09;-1.85986777702161e-09 7.82540023894543e-09 -1.8957321828871e-09;-1.7901190036642e-09 -1.8957321828871e-09 7.91264394645417e-09]  x1=[139.593565234006 4223.2246870777 4223.34301290055;314.159265358979 314.159265358979 314.159265358979;0.93049120516093 1.89139243776416 -2.81971500203384]  x2=[139.596827955923 4222.34183377535 4222.45832100252;314.159265358979 314.159265358979 314.159265358979;0.930538259653429 1.89128639160062 -2.81981974944059]  x3=[0.135987367536833 6.25139247202186 6.32939138956456;314.159265358979 314.159265358979 314.159265358979;0.924773461220038 2.03699553491578 -2.67375446041921]  x4=[0.10808998359841 15.3280702332523 15.4174543796233;314.159265358979 314.159265358979 314.159265358979;0.937261954609327 1.83187520507369 -2.87976923231697]  x5=1.34151653007687e-06  V1=ones(3,3)  V2=ones(3,3)  I1=ones(3,3)  I2=ones(3,3)  nHarmo=1  Measurements=None  Decoupling=off  VsMag0=0  VrMag0=0  VsAngle0=0  VrAngle0=0  IsMag0=0  IrMag0=0  IsAngle0=0  IrAngle0=0
      settings: SourceProductBaseCode=PS
  Line 3 : spsDistributedParametersLineLib/Distributed Parameters Line  Phases=3  Length=0.28003  Frequency=50  Resistance=[0.476003738225748 0.351747138225748 0.351747138225748;0.351747138225748 0.476003738225748 0.351747138225748;0.351747138225748 0.351747138225748 0.476003738225748]  Inductance=[0.000705954362986426 0.000459934243504405 0.000459934243504405;0.000459934243504405 0.000705954362986426 0.000459934243504405;0.000459934243504405 0.000459934243504405 0.000705954362986426]  Capacitance=[5.7561313269996e-07 -1.37543883484145e-07 -1.37543912800485e-07;-1.37543883484145e-07 5.75613027339387e-07 -1.37543875208088e-07;-1.37543912800485e-07 -1.37543875208088e-07 5.75613005057695e-07]  x1=[87.2784474669042 4217.75377370591 4217.44930563501;314.159265358979 314.159265358979 314.159265358979;1.07714915979928 1.80783649231744 -2.9034758566981]  x2=[87.2786300461154 4217.75686845333 4217.45240278323;314.159265358979 314.159265358979 314.159265358979;1.0771440619415 1.80783531251349 -2.90347703713064]  x3=[1.18260582710926 226.766358600512 226.749991751986;314.159265358979 314.159265358979 314.159265358979;1.07504862288657 1.80662354393233 -2.90468919605049]  x4=[1.18265706398664 226.766378331968 226.749971140506;314.159265358979 314.159265358979 314.159265358979;1.07729776135001 1.80788242963964 -2.90342952883494]  x5=6.18987206366653e-06  V1=ones(3,3)  V2=ones(3,3)  I1=ones(3,3)  I2=ones(3,3)  nHarmo=1  Measurements=None  Decoupling=off  VsMag0=0  VrMag0=0  VsAngle0=0  VrAngle0=0  IsMag0=0  IrMag0=0  IsAngle0=0  IrAngle0=0
      settings: SourceProductBaseCode=PS
  Line 30 : spsDistributedParametersLineLib/Distributed Parameters Line  Phases=3  Length=1.11  Frequency=50  Resistance=[0.502970710632245 0.0486237908083191 0.0486712220507153;0.0486237908083191 0.502875844822084 0.0486237934466192;0.0486712220507153 0.0486237934466192 0.502970710632245]  Inductance=[0.00286900545038753 0.00133270803418135 0.00132951476746136;0.00133270803418135 0.00286931445999602 0.00133799988507366;0.00132951476746136 0.00133799988507366 0.00286900545038753]  Capacitance=[8.11484299003193e-09 -1.94249816214699e-09 -1.86930692621136e-09;-1.94249816214699e-09 8.0425699231653e-09 -1.98049571960044e-09;-1.86930692621136e-09 -1.98049571960044e-09 8.13337738722527e-09]  x1=[174.117109770187 2390.94189935978 2394.61464486616;314.159265358979 314.159265358979 314.159265358979;0.849468685913811 -0.860439668129714 -2.42962031247911]  x2=[174.117358023186 2390.94413526641 2394.61688925047;314.159265358979 314.159265358979 314.159265358979;0.84946819370226 -0.860440545931823 -2.42962119784236]  x3=[0.152647233351537 6.08204000336836 6.13815396542189;314.159265358979 314.159265358979 314.159265358979;0.847779783441453 -0.861807701125025 -2.4309898883284]  x4=[0.152647233388058 6.08204000521585 6.13815396727617;314.159265358979 314.159265358979 314.159265358979;0.849468193740857 -0.860440545928679 -2.42962119784054]  x5=5.37516004033389e-06  V1=ones(3,3)  V2=ones(3,3)  I1=ones(3,3)  I2=ones(3,3)  nHarmo=1  Measurements=None  Decoupling=off  VsMag0=0  VrMag0=0  VsAngle0=0  VrAngle0=0  IsMag0=0  IrMag0=0  IsAngle0=0  IrAngle0=0
      settings: SourceProductBaseCode=PS
  Line 31 : spsDistributedParametersLineLib/Distributed Parameters Line  Phases=3  Length=0.02  Frequency=50  Resistance=[0.646656091154803 0.0486237908083191 0.0486712220507153;0.0486237908083191 0.646561225344642 0.0486237934466192;0.0486712220507153 0.0486237934466192 0.646656091154803]  Inductance=[0.00282448912315926 0.00133270803418135 0.00132951476746136;0.00133270803418135 0.00282479813276775 0.00133799988507366;0.00132951476746136 0.00133799988507366 0.00282448912315926]  Capacitance=[7.89543174552926e-09 -1.85986777702161e-09 -1.7901190036642e-09;-1.85986777702161e-09 7.82540023894543e-09 -1.8957321828871e-09;-1.7901190036642e-09 -1.8957321828871e-09 7.91264394645417e-09]  x1=[153.230127998546 2391.27414651659 2395.46660308653;314.159265358979 314.159265358979 314.159265358979;0.938142925866437 -0.865115597320735 -2.43425839069254]  x2=[153.230370640917 2391.26534326387 2395.45779665592;314.159265358979 314.159265358979 314.159265358979;0.938142605420199 -0.865117419435394 -2.43426019857906]  x3=[0.135487350546719 5.45487548693329 5.51115286887288;314.159265358979 314.159265358979 314.159265358979;0.890427877735878 -0.840847288884499 -2.41026567975298]  x4=[0.132770538398918 6.7187980916648 6.7774647021665;314.159265358979 314.159265358979 314.159265358979;0.986804367458558 -0.88484127342735 -2.45379097418423]  x5=9.5829454252223e-08  V1=ones(3,3)  V2=ones(3,3)  I1=ones(3,3)  I2=ones(3,3)  nHarmo=1  Measurements=None  Decoupling=off  VsMag0=0  VrMag0=0  VsAngle0=0  VrAngle0=0  IsMag0=0  IrMag0=0  IsAngle0=0  IrAngle0=0
      settings: SourceProductBaseCode=PS
  Line 32 : spsDistributedParametersLineLib/Distributed Parameters Line  Phases=3  Length=1.15  Frequency=50  Resistance=[0.646656091154803 0.0486237908083191 0.0486712220507153;0.0486237908083191 0.646561225344642 0.0486237934466192;0.0486712220507153 0.0486237934466192 0.646656091154803]  Inductance=[0.00282448912315926 0.00133270803418135 0.00132951476746136;0.00133270803418135 0.00282479813276775 0.00133799988507366;0.00132951476746136 0.00133799988507366 0.00282448912315926]  Capacitance=[7.89543174552926e-09 -1.85986777702161e-09 -1.7901190036642e-09;-1.85986777702161e-09 7.82540023894543e-09 -1.8957321828871e-09;-1.7901190036642e-09 -1.8957321828871e-09 7.91264394645417e-09]  x1=[153.230127998546 2391.27414651659 2395.46660308653;314.159265358979 314.159265358979 314.159265358979;0.936441953197896 -0.866466908389391 -2.43561098811364]  x2=[153.233923966048 2390.86248388167 2395.05514626126;314.159265358979 314.159265358979 314.159265358979;0.936435010504987 -0.866498451899493 -2.43564199996079]  x3=[0.134157315855614 5.65874582422695 5.71522501268418;314.159265358979 314.159265358979 314.159265358979;0.922075894467933 -0.827806112795469 -2.39731679464492]  x4=[0.133669524037514 6.50350854249352 6.5616659890612;314.159265358979 314.159265358979 314.159265358979;0.949118924044183 -0.901419739156289 -2.47028056162485]  x5=5.51019361950282e-06  V1=ones(3,3)  V2=ones(3,3)  I1=ones(3,3)  I2=ones(3,3)  nHarmo=1  Measurements=None  Decoupling=off  VsMag0=0  VrMag0=0  VsAngle0=0  VrAngle0=0  IsMag0=0  IrMag0=0  IsAngle0=0  IrAngle0=0
      settings: SourceProductBaseCode=PS
  Line 33 : spsDistributedParametersLineLib/Distributed Parameters Line  Phases=3  Length=0.18999  Frequency=50  Resistance=[0.646656091154803 0.0486237908083191 0.0486712220507153;0.0486237908083191 0.646561225344642 0.0486237934466192;0.0486712220507153 0.0486237934466192 0.646656091154803]  Inductance=[0.00282448912315926 0.00133270803418135 0.00132951476746136;0.00133270803418135 0.00282479813276775 0.00133799988507366;0.00132951476746136 0.00133799988507366 0.00282448912315926]  Capacitance=[7.89543174552926e-09 -1.85986777702161e-09 -1.7901190036642e-09;-1.85986777702161e-09 7.82540023894543e-09 -1.8957321828871e-09;-1.7901190036642e-09 -1.8957321828871e-09 7.91264394645417e-09]  x1=[153.233923966048 2390.86248388167 2395.05514626126;314.159265358979 314.159265358979 314.159265358979;0.937880099683329 -0.865350423457882 -2.43449287867739]  x2=[153.23410399113 2390.83743582921 2395.03011364573;314.159265358979 314.159265358979 314.159265358979;0.937879732574347 -0.865351400185327 -2.43449382349532]  x3=[0.134021612128501 5.93762545616558 5.99478691217682;314.159265358979 314.159265358979 314.159265358979;0.933808116214242 -0.849565080741354 -2.41883991758179]  x4=[0.133911387204022 6.23010379991839 6.28785505037653;314.159265358979 314.159265358979 314.159265358979;0.941668951903914 -0.880617485621142 -2.44963927552907]  x5=9.10331900668992e-07  V1=ones(3,3)  V2=ones(3,3)  I1=ones(3,3)  I2=ones(3,3)  nHarmo=1  Measurements=None  Decoupling=off  VsMag0=0  VrMag0=0  VsAngle0=0  VrAngle0=0  IsMag0=0  IrMag0=0  IsAngle0=0  IrAngle0=0
      settings: SourceProductBaseCode=PS
  Line 34 : spsDistributedParametersLineLib/Distributed Parameters Line  Phases=3  Length=0.34002  Frequency=50  Resistance=[0.646656091154803 0.0486237908083191 0.0486712220507153;0.0486237908083191 0.646561225344642 0.0486237934466192;0.0486712220507153 0.0486237934466192 0.646656091154803]  Inductance=[0.00282448912315926 0.00133270803418135 0.00132951476746136;0.00133270803418135 0.00282479813276775 0.00133799988507366;0.00132951476746136 0.00133799988507366 0.00282448912315926]  Capacitance=[7.89543174552926e-09 -1.85986777702161e-09 -1.7901190036642e-09;-1.85986777702161e-09 7.82540023894543e-09 -1.8957321828871e-09;-1.7901190036642e-09 -1.8957321828871e-09 7.91264394645417e-09]  x1=[153.233923966048 2390.86248388167 2395.05514626126;314.159265358979 314.159265358979 314.159265358979;0.937654261692655 -0.865529836908882 -2.4346724629173]  x2=[153.234624964005 2390.78461941079 2394.97731142616;314.159265358979 314.159265358979 314.159265358979;0.937653145104761 -0.865536897499382 -2.43467941898661]  x3=[0.134149496175836 5.80661770596711 5.86350238542297;314.159265358979 314.159265358979 314.159265358979;0.929080532757777 -0.842538209878846 -2.41189216195786]  x4=[0.133771618235119 6.3604177378356 6.41839502912858;314.159265358979 314.159265358979 314.159265358979;0.945738513686327 -0.886914986725278 -2.4558791342442]  x5=1.62919655174204e-06  V1=ones(3,3)  V2=ones(3,3)  I1=ones(3,3)  I2=ones(3,3)  nHarmo=1  Measurements=None  Decoupling=off  VsMag0=0  VrMag0=0  VsAngle0=0  VrAngle0=0  IsMag0=0  IrMag0=0  IsAngle0=0  IrAngle0=0
      settings: SourceProductBaseCode=PS
  Line 35 : spsDistributedParametersLineLib/Distributed Parameters Line  Phases=3  Length=0.12001  Frequency=50  Resistance=[0.646656091154803 0.0486237908083191 0.0486712220507153;0.0486237908083191 0.646561225344642 0.0486237934466192;0.0486712220507153 0.0486237934466192 0.646656091154803]  Inductance=[0.00282448912315926 0.00133270803418135 0.00132951476746136;0.00133270803418135 0.00282479813276775 0.00133799988507366;0.00132951476746136 0.00133799988507366 0.00282448912315926]  Capacitance=[7.89543174552926e-09 -1.85986777702161e-09 -1.7901190036642e-09;-1.85986777702161e-09 7.82540023894543e-09 -1.8957321828871e-09;-1.7901190036642e-09 -1.8957321828871e-09 7.91264394645417e-09]  x1=[153.234624964005 2390.78461941079 2394.97731142616;314.159265358979 314.159265358979 314.159265358979;0.937984322978041 -0.865273798430165 -2.4344160694657]  x2=[153.234723381387 2390.77095103028 2394.96365022423;314.159265358979 314.159265358979 314.159265358979;0.937984143886448 -0.865274504167284 -2.43441675729628]  x3=[0.134032568727206 5.95478629795986 6.01199252804239;314.159265358979 314.159265358979 314.159265358979;0.93453723277752 -0.852246304782311 -2.42149761720487]  x4=[0.1339101534125 6.21308203810098 6.27080554573555;314.159265358979 314.159265358979 314.159265358979;0.941253649790315 -0.877900900711225 -2.4469426804373]  x5=5.75024640240464e-07  V1=ones(3,3)  V2=ones(3,3)  I1=ones(3,3)  I2=ones(3,3)  nHarmo=1  Measurements=None  Decoupling=off  VsMag0=0  VrMag0=0  VsAngle0=0  VrAngle0=0  IsMag0=0  IrMag0=0  IsAngle0=0  IrAngle0=0
      settings: SourceProductBaseCode=PS
  Line 36 : spsDistributedParametersLineLib/Distributed Parameters Line  Phases=3  Length=0.82  Frequency=50  Resistance=[0.646656091154803 0.0486237908083191 0.0486712220507153;0.0486237908083191 0.646561225344642 0.0486237934466192;0.0486712220507153 0.0486237934466192 0.646656091154803]  Inductance=[0.00282448912315926 0.00133270803418135 0.00132951476746136;0.00133270803418135 0.00282479813276775 0.00133799988507366;0.00132951476746136 0.00133799988507366 0.00282448912315926]  Capacitance=[7.89543174552926e-09 -1.85986777702161e-09 -1.7901190036642e-09;-1.85986777702161e-09 7.82540023894543e-09 -1.8957321828871e-09;-1.7901190036642e-09 -1.8957321828871e-09 7.91264394645417e-09]  x1=[153.234624964005 2390.78461941079 2394.97731142616;314.159265358979 314.159265358979 314.159265358979;0.936930638147729 -0.866110881823925 -2.43525394970358]  x2=[153.235460823007 2390.68843849365 2394.88114635184;314.159265358979 314.159265358979 314.159265358979;0.936929681896354 -0.866122133324562 -2.43526506339407]  x3=[0.134054086184571 5.93104397380724 5.98814009724907;314.159265358979 314.159265358979 314.159265358979;0.932309381950793 -0.85626740757645 -2.42550350750748]  x4=[0.133798673317231 6.22652032700826 6.28418896890224;314.159265358979 314.159265358979 314.159265358979;0.940324082190587 -0.876455836197233 -2.44551459543654]  x5=3.92900762434114e-06  V1=ones(3,3)  V2=ones(3,3)  I1=ones(3,3)  I2=ones(3,3)  nHarmo=1  Measurements=None  Decoupling=off  VsMag0=0  VrMag0=0  VsAngle0=0  VrAngle0=0  IsMag0=0  IrMag0=0  IsAngle0=0  IrAngle0=0
      settings: SourceProductBaseCode=PS
  Line 37 : spsDistributedParametersLineLib/Distributed Parameters Line  Phases=3  Length=1.11  Frequency=50  Resistance=[0.646656091154803 0.0486237908083191 0.0486712220507153;0.0486237908083191 0.646561225344642 0.0486237934466192;0.0486712220507153 0.0486237934466192 0.646656091154803]  Inductance=[0.00282448912315926 0.00133270803418135 0.00132951476746136;0.00133270803418135 0.00282479813276775 0.00133799988507366;0.00132951476746136 0.00133799988507366 0.00282448912315926]  Capacitance=[7.89543174552926e-09 -1.85986777702161e-09 -1.7901190036642e-09;-1.85986777702161e-09 7.82540023894543e-09 -1.8957321828871e-09;-1.7901190036642e-09 -1.8957321828871e-09 7.91264394645417e-09]  x1=[153.212558124091 2392.15576627603 2396.34818431214;314.159265358979 314.159265358979 314.159265358979;0.936527890210652 -0.866285253189953 -2.43543057006674]  x2=[153.230127998546 2391.27414651659 2395.46660308653;314.159265358979 314.159265358979 314.159265358979;0.936502164619791 -0.866419074369261 -2.43556310855891]  x3=[0.135763387573611 5.03716609743806 5.09238086398861;314.159265358979 314.159265358979 314.159265358979;0.873057883964176 -0.798128681550033 -2.36804348064367]  x4=[0.132564158465786 7.14110155666708 7.20041308134237;314.159265358979 314.159265358979 314.159265358979;0.999814325991861 -0.915588397773758 -2.48431817500408]  x5=5.31853471099837e-06  V1=ones(3,3)  V2=ones(3,3)  I1=ones(3,3)  I2=ones(3,3)  nHarmo=1  Measurements=None  Decoupling=off  VsMag0=0  VrMag0=0  VsAngle0=0  VrAngle0=0  IsMag0=0  IrMag0=0  IsAngle0=0  IrAngle0=0
      settings: SourceProductBaseCode=PS
  Line 38 : spsDistributedParametersLineLib/Distributed Parameters Line  Phases=3  Length=0.20999  Frequency=50  Resistance=[0.646656091154803 0.0486237908083191 0.0486712220507153;0.0486237908083191 0.646561225344642 0.0486237934466192;0.0486712220507153 0.0486237934466192 0.646656091154803]  Inductance=[0.00282448912315926 0.00133270803418135 0.00132951476746136;0.00133270803418135 0.00282479813276775 0.00133799988507366;0.00132951476746136 0.00133799988507366 0.00282448912315926]  Capacitance=[7.89543174552926e-09 -1.85986777702161e-09 -1.7901190036642e-09;-1.85986777702161e-09 7.82540023894543e-09 -1.8957321828871e-09;-1.7901190036642e-09 -1.8957321828871e-09 7.91264394645417e-09]  x1=[153.212558124091 2392.15576627603 2396.34818431214;314.159265358979 314.159265358979 314.159265358979;0.937882662256151 -0.865208975778536 -2.43435326811544]  x2=[153.213590781307 2392.16800458541 2396.36036495859;314.159265358979 314.159265358979 314.159265358979;0.937881616648445 -0.865215489481055 -2.43435977773203]  x3=[0.134635296009935 6.08755259574682 6.14506938403262;314.159265358979 314.159265358979 314.159265358979;0.91863993031571 -0.88571531736767 -2.45470042474449]  x4=[0.133305690867782 6.08763682984433 6.1450721673001;314.159265358979 314.159265358979 314.159265358979;0.956998613740082 -0.844960566613944 -2.41426400619753]  x5=1.00616135492121e-06  V1=ones(3,3)  V2=ones(3,3)  I1=ones(3,3)  I2=ones(3,3)  nHarmo=1  Measurements=None  Decoupling=off  VsMag0=0  VrMag0=0  VsAngle0=0  VrAngle0=0  IsMag0=0  IrMag0=0  IsAngle0=0  IrAngle0=0
      settings: SourceProductBaseCode=PS
  Line 39 : spsDistributedParametersLineLib/Distributed Parameters Line  Phases=3  Length=0.23002  Frequency=50  Resistance=[0.476003738225748 0.351747138225748 0.351747138225748;0.351747138225748 0.476003738225748 0.351747138225748;0.351747138225748 0.351747138225748 0.476003738225748]  Inductance=[0.000705954362986426 0.000459934243504405 0.000459934243504405;0.000459934243504405 0.000705954362986426 0.000459934243504405;0.000459934243504405 0.000459934243504405 0.000705954362986426]  Capacitance=[5.7561313269996e-07 -1.37543883484145e-07 -1.37543912800485e-07;-1.37543883484145e-07 5.75613027339387e-07 -1.37543875208088e-07;-1.37543912800485e-07 -1.37543875208088e-07 5.75613005057695e-07]  x1=[128.937995458432 2392.16649760036 2396.88280688884;314.159265358979 314.159265358979 314.159265358979;1.07459563368783 -0.784215908326795 -2.35345677130392]  x2=[128.938159946897 2392.16759344276 2396.88390489159;314.159265358979 314.159265358979 314.159265358979;1.07459268770877 -0.784216644798089 -2.3534575077751]  x3=[1.7481716507325 128.646408466006 128.900033137136;314.159265358979 314.159265358979 314.159265358979;1.07299683828971 -0.78517345599754 -2.35441431889997]  x4=[1.74817165276613 128.646408488778 128.900033160072;314.159265358979 314.159265358979 314.159265358979;1.07459268770351 -0.784216644798272 -2.35345750777576]  x5=5.08443513939426e-06  V1=ones(3,3)  V2=ones(3,3)  I1=ones(3,3)  I2=ones(3,3)  nHarmo=1  Measurements=None  Decoupling=off  VsMag0=0  VrMag0=0  VsAngle0=0  VrAngle0=0  IsMag0=0  IrMag0=0  IsAngle0=0  IrAngle0=0
      settings: SourceProductBaseCode=PS
  Line 4 : spsDistributedParametersLineLib/Distributed Parameters Line  Phases=3  Length=0.28003  Frequency=50  Resistance=[0.646656091154803 0.0486237908083191 0.0486712220507153;0.0486237908083191 0.646561225344642 0.0486237934466192;0.0486712220507153 0.0486237934466192 0.646656091154803]  Inductance=[0.00282448912315926 0.00133270803418135 0.00132951476746136;0.00133270803418135 0.00282479813276775 0.00133799988507366;0.00132951476746136 0.00133799988507366 0.00282448912315926]  Capacitance=[7.89543174552926e-09 -1.85986777702161e-09 -1.7901190036642e-09;-1.85986777702161e-09 7.82540023894543e-09 -1.8957321828871e-09;-1.7901190036642e-09 -1.8957321828871e-09 7.91264394645417e-09]  x1=[139.624133846896 4217.05249779218 4217.15010477417;314.159265358979 314.159265358979 314.159265358979;0.930858418144753 1.89028560487824 -2.82081161413781]  x2=[139.624195099916 4217.05366845318 4217.15127755993;314.159265358979 314.159265358979 314.159265358979;0.93085822933126 1.89028525169055 -2.82081197029047]  x3=[0.122061806521893 10.7285123386744 10.8111375362311;314.159265358979 314.159265358979 314.159265358979;0.929607181287013 1.88928910023914 -2.82180899896606]  x4=[0.122061623032824 10.7285121401494 10.8111377478062;314.159265358979 314.159265358979 314.159265358979;0.931687923467966 1.8909468466586 -2.82014981424203]  x5=1.3417561037125e-06  V1=ones(3,3)  V2=ones(3,3)  I1=ones(3,3)  I2=ones(3,3)  nHarmo=1  Measurements=None  Decoupling=off  VsMag0=0  VrMag0=0  VsAngle0=0  VrAngle0=0  IsMag0=0  IrMag0=0  IsAngle0=0  IrAngle0=0
      settings: SourceProductBaseCode=PS
  Line 40 : spsDistributedParametersLineLib/Distributed Parameters Line  Phases=3  Length=0.24  Frequency=50  Resistance=[0.646656091154803 0.0486237908083191 0.0486712220507153;0.0486237908083191 0.646561225344642 0.0486237934466192;0.0486712220507153 0.0486237934466192 0.646656091154803]  Inductance=[0.00282448912315926 0.00133270803418135 0.00132951476746136;0.00133270803418135 0.00282479813276775 0.00133799988507366;0.00132951476746136 0.00133799988507366 0.00282448912315926]  Capacitance=[7.89543174552926e-09 -1.85986777702161e-09 -1.7901190036642e-09;-1.85986777702161e-09 7.82540023894543e-09 -1.8957321828871e-09;-1.7901190036642e-09 -1.8957321828871e-09 7.91264394645417e-09]  x1=[153.209700726879 2392.33280691669 2396.52386758149;314.159265358979 314.159265358979 314.159265358979;0.937849540955194 -0.865207977096836 -2.43435252492661]  x2=[153.212558124086 2392.15576627611 2396.34818431222;314.159265358979 314.159265358979 314.159265358979;0.937837488636867 -0.865244863252122 -2.43438918975136]  x3=[0.132898075555068 5.03002807748298 5.0908406195725;314.159265358979 314.159265358979 314.159265358979;0.881538864807227 -0.821771427937942 -2.39256728749263]  x4=[0.135400951927345 7.15077743499702 7.20442623317237;314.159265358979 314.159265358979 314.159265358979;0.992748373434902 -0.89603325826109 -2.46415118539181]  x5=1.14995345102668e-06  V1=ones(3,3)  V2=ones(3,3)  I1=ones(3,3)  I2=ones(3,3)  nHarmo=1  Measurements=None  Decoupling=off  VsMag0=0  VrMag0=0  VsAngle0=0  VrAngle0=0  IsMag0=0  IrMag0=0  IsAngle0=0  IrAngle0=0
      settings: SourceProductBaseCode=PS
  Line 41 : spsDistributedParametersLineLib/Distributed Parameters Line  Phases=3  Length=0.03  Frequency=50  Resistance=[0.476003738225748 0.351747138225748 0.351747138225748;0.351747138225748 0.476003738225748 0.351747138225748;0.351747138225748 0.351747138225748 0.476003738225748]  Inductance=[0.000705954362986426 0.000459934243504405 0.000459934243504405;0.000459934243504405 0.000705954362986426 0.000459934243504405;0.000459934243504405 0.000459934243504405 0.000705954362986426]  Capacitance=[5.7561313269996e-07 -1.37543883484145e-07 -1.37543912800485e-07;-1.37543883484145e-07 5.75613027339387e-07 -1.37543875208088e-07;-1.37543912800485e-07 -1.37543875208088e-07 5.75613005057695e-07]  x1=[128.988731614043 2390.89852283072 2395.61456770164;314.159265358979 314.159265358979 314.159265358979;1.07585331541723 -0.783647737033645 -2.35288668623118]  x2=[128.988736171231 2390.89856079886 2395.61460585816;314.159265358979 314.159265358979 314.159265358979;1.07585319347413 -0.783647762530372 -2.35288671186124]  x3=[1.75301529039677 128.707268861607 128.961117386385;314.159265358979 314.159265358979 314.159265358979;1.07550887093704 -0.783837251426574 -2.35307678559337]  x4=[1.75312252914097 128.707249510834 128.96113094774;314.159265358979 314.159265358979 314.159265358979;1.07598926988593 -0.783583093016753 -2.35282145740353]  x5=6.63129528657629e-07  V1=ones(3,3)  V2=ones(3,3)  I1=ones(3,3)  I2=ones(3,3)  nHarmo=1  Measurements=None  Decoupling=off  VsMag0=0  VrMag0=0  VsAngle0=0  VrAngle0=0  IsMag0=0  IrMag0=0  IsAngle0=0  IrAngle0=0
      settings: SourceProductBaseCode=PS
  Line 42 : spsDistributedParametersLineLib/Distributed Parameters Line  Phases=3  Length=0.02  Frequency=50  Resistance=[0.646656091154803 0.0486237908083191 0.0486712220507153;0.0486237908083191 0.646561225344642 0.0486237934466192;0.0486712220507153 0.0486237934466192 0.646656091154803]  Inductance=[0.00282448912315926 0.00133270803418135 0.00132951476746136;0.00133270803418135 0.00282479813276775 0.00133799988507366;0.00132951476746136 0.00133799988507366 0.00282448912315926]  Capacitance=[7.89543174552926e-09 -1.85986777702161e-09 -1.7901190036642e-09;-1.85986777702161e-09 7.82540023894543e-09 -1.8957321828871e-09;-1.7901190036642e-09 -1.8957321828871e-09 7.91264394645417e-09]  x1=[153.209700726879 2392.33280691669 2396.52386758149;314.159265358979 314.159265358979 314.159265358979;0.938180703775618 -0.864944889986124 -2.4340891873756]  x2=[153.209713890097 2392.33103545463 2396.52209633678;314.159265358979 314.159265358979 314.159265358979;0.938180692162723 -0.864945083941827 -2.43408937873265]  x3=[0.134051172363834 5.97784828880328 6.03513852751897;314.159265358979 314.159265358979 314.159265358979;0.935620903319396 -0.856929128719586 -2.42614145383634]  x4=[0.133860294898411 6.19869643869784 6.25641614231707;314.159265358979 314.159265358979 314.159265358979;0.940714015320332 -0.872698740237325 -2.44177952354658]  x5=9.5829454252223e-08  V1=ones(3,3)  V2=ones(3,3)  I1=ones(3,3)  I2=ones(3,3)  nHarmo=1  Measurements=None  Decoupling=off  VsMag0=0  VrMag0=0  VsAngle0=0  VrAngle0=0  IsMag0=0  IrMag0=0  IsAngle0=0  IrAngle0=0
      settings: SourceProductBaseCode=PS
  Line 43 : spsDistributedParametersLineLib/Distributed Parameters Line  Phases=3  Length=0.5  Frequency=50  Resistance=[0.646656091154803 0.0486237908083191 0.0486712220507153;0.0486237908083191 0.646561225344642 0.0486237934466192;0.0486712220507153 0.0486237934466192 0.646656091154803]  Inductance=[0.00282448912315926 0.00133270803418135 0.00132951476746136;0.00133270803418135 0.00282479813276775 0.00133799988507366;0.00132951476746136 0.00133799988507366 0.00282448912315926]  Capacitance=[7.89543174552926e-09 -1.85986777702161e-09 -1.7901190036642e-09;-1.85986777702161e-09 7.82540023894543e-09 -1.8957321828871e-09;-1.7901190036642e-09 -1.8957321828871e-09 7.91264394645417e-09]  x1=[153.203352849777 2392.74528951814 2396.93351438967;314.159265358979 314.159265358979 314.159265358979;0.937483753216874 -0.865436877301409 -2.43458224395416]  x2=[153.209700726879 2392.33280691669 2396.52386758149;314.159265358979 314.159265358979 314.159265358979;0.937458166712875 -0.865518898227677 -2.43466374203235]  x3=[0.132996455190241 4.921388055176 4.98187180105692;314.159265358979 314.159265358979 314.159265358979;0.877876508233487 -0.812025935079932 -2.38297564891433]  x4=[0.135308264129347 7.26108829843137 7.31487683564196;314.159265358979 314.159265358979 314.159265358979;0.995299782557578 -0.902198507428082 -2.47029255424995]  x5=2.39573635630557e-06  V1=ones(3,3)  V2=ones(3,3)  I1=ones(3,3)  I2=ones(3,3)  nHarmo=1  Measurements=None  Decoupling=off  VsMag0=0  VrMag0=0  VsAngle0=0  VrAngle0=0  IsMag0=0  IrMag0=0  IsAngle0=0  IrAngle0=0
      settings: SourceProductBaseCode=PS
  Line 44 : spsDistributedParametersLineLib/Distributed Parameters Line  Phases=3  Length=1.11  Frequency=50  Resistance=[0.502970710632245 0.0486237908083191 0.0486712220507153;0.0486237908083191 0.502875844822084 0.0486237934466192;0.0486712220507153 0.0486237934466192 0.502970710632245]  Inductance=[0.00286900545038753 0.00133270803418135 0.00132951476746136;0.00133270803418135 0.00286931445999602 0.00133799988507366;0.00132951476746136 0.00133799988507366 0.00286900545038753]  Capacitance=[8.11484299003193e-09 -1.94249816214699e-09 -1.86930692621136e-09;-1.94249816214699e-09 8.0425699231653e-09 -1.98049571960044e-09;-1.86930692621136e-09 -1.98049571960044e-09 8.13337738722527e-09]  x1=[174.084755739478 2396.11508208311 2399.77223791544;314.159265358979 314.159265358979 314.159265358979;0.849577928274968 -0.859530793740428 -2.42871828913589]  x2=[174.08500394633 2396.11732282742 2399.77448713379;314.159265358979 314.159265358979 314.159265358979;0.84957743606373 -0.859531671542514 -2.42871917449917]  x3=[0.152618868825002 6.09519946335855 6.15137450600136;314.159265358979 314.159265358979 314.159265358979;0.847889025907192 -0.86089882671792 -2.43008786499985]  x4=[0.152618868816897 6.09519946521337 6.15137450797948;314.159265358979 314.159265358979 314.159265358979;0.849577435994565 -0.859531671557247 -2.42871917448271]  x5=5.37516004033389e-06  V1=ones(3,3)  V2=ones(3,3)  I1=ones(3,3)  I2=ones(3,3)  nHarmo=1  Measurements=None  Decoupling=off  VsMag0=0  VrMag0=0  VsAngle0=0  VrAngle0=0  IsMag0=0  IrMag0=0  IsAngle0=0  IrAngle0=0
      settings: SourceProductBaseCode=PS
  Line 45 : spsDistributedParametersLineLib/Distributed Parameters Line  Phases=3  Length=0.03  Frequency=50  Resistance=[0.476003738225748 0.351747138225748 0.351747138225748;0.351747138225748 0.476003738225748 0.351747138225748;0.351747138225748 0.351747138225748 0.476003738225748]  Inductance=[0.000705954362986426 0.000459934243504405 0.000459934243504405;0.000459934243504405 0.000705954362986426 0.000459934243504405;0.000459934243504405 0.000459934243504405 0.000705954362986426]  Capacitance=[5.7561313269996e-07 -1.37543883484145e-07 -1.37543912800485e-07;-1.37543883484145e-07 5.75613027339387e-07 -1.37543875208088e-07;-1.37543912800485e-07 -1.37543875208088e-07 5.75613005057695e-07]  x1=[128.837965700403 2396.07271829091 2400.77259937988;314.159265358979 314.159265358979 314.159265358979;1.07641786297578 -0.782739641086843 -2.35198399079567]  x2=[128.837970249233 2396.07275634118 2400.77263761849;314.159265358979 314.159265358979 314.159265358979;1.07641774096466 -0.782739666583583 -2.3519840164257]  x3=[1.75096615097623 128.985807049813 129.238785392142;314.159265358979 314.159265358979 314.159265358979;1.07607331724176 -0.78292915549521 -2.35217408995823]  x4=[1.75107358911746 128.985787676827 129.238798990405;314.159265358979 314.159265358979 314.159265358979;1.0765539186059 -0.782674997054493 -2.35191876216735]  x5=6.63129528657629e-07  V1=ones(3,3)  V2=ones(3,3)  I1=ones(3,3)  I2=ones(3,3)  nHarmo=1  Measurements=None  Decoupling=off  VsMag0=0  VrMag0=0  VsAngle0=0  VrAngle0=0  IsMag0=0  IrMag0=0  IsAngle0=0  IrAngle0=0
      settings: SourceProductBaseCode=PS
  Line 46 : spsDistributedParametersLineLib/Distributed Parameters Line  Phases=3  Length=0.28003  Frequency=50  Resistance=[0.476003738225748 0.351747138225748 0.351747138225748;0.351747138225748 0.476003738225748 0.351747138225748;0.351747138225748 0.351747138225748 0.476003738225748]  Inductance=[0.000705954362986426 0.000459934243504405 0.000459934243504405;0.000459934243504405 0.000705954362986426 0.000459934243504405;0.000459934243504405 0.000459934243504405 0.000705954362986426]  Capacitance=[5.7561313269996e-07 -1.37543883484145e-07 -1.37543912800485e-07;-1.37543883484145e-07 5.75613027339387e-07 -1.37543875208088e-07;-1.37543912800485e-07 -1.37543875208088e-07 5.75613005057695e-07]  x1=[128.837965700403 2396.07271829091 2400.77259937988;314.159265358979 314.159265358979 314.159265358979;1.07468158560115 -0.78378008789209 -2.35302443752048]  x2=[128.838052814648 2395.97068171338 2400.67066906338;314.159265358979 314.159265358979 314.159265358979;1.07465507302118 -0.783791963772372 -2.35303637463203]  x3=[1.74225348008066 126.346934175727 126.599167456367;314.159265358979 314.159265358979 314.159265358979;1.06866383389768 -0.778637173462468 -2.34793690767294]  x4=[1.74931976431486 131.299884698145 131.552942365902;314.159265358979 314.159265358979 314.159265358979;1.0787057128987 -0.78988449071425 -2.35907598138563]  x5=6.18987206366653e-06  V1=ones(3,3)  V2=ones(3,3)  I1=ones(3,3)  I2=ones(3,3)  nHarmo=1  Measurements=None  Decoupling=off  VsMag0=0  VrMag0=0  VsAngle0=0  VrAngle0=0  IsMag0=0  IrMag0=0  IsAngle0=0  IrAngle0=0
      settings: SourceProductBaseCode=PS
  Line 47 : spsDistributedParametersLineLib/Distributed Parameters Line  Phases=3  Length=0.28003  Frequency=50  Resistance=[0.646656091154803 0.0486237908083191 0.0486712220507153;0.0486237908083191 0.646561225344642 0.0486237934466192;0.0486712220507153 0.0486237934466192 0.646656091154803]  Inductance=[0.00282448912315926 0.00133270803418135 0.00132951476746136;0.00133270803418135 0.00282479813276775 0.00133799988507366;0.00132951476746136 0.00133799988507366 0.00282448912315926]  Capacitance=[7.89543174552926e-09 -1.85986777702161e-09 -1.7901190036642e-09;-1.85986777702161e-09 7.82540023894543e-09 -1.8957321828871e-09;-1.7901190036642e-09 -1.8957321828871e-09 7.91264394645417e-09]  x1=[153.159179485536 2395.97158224862 2400.14761691967;314.159265358979 314.159265358979 314.159265358979;0.937946677145248 -0.864666615998529 -2.43381602702545]  x2=[153.16626200144 2395.45047998511 2399.62815160235;314.159265358979 314.159265358979 314.159265358979;0.93792760278599 -0.864746907831608 -2.43389561336886]  x3=[0.134920535448977 3.70157273482948 3.75743092438561;314.159265358979 314.159265358979 314.159265358979;0.829392992227737 -0.646572802886826 -2.22050446008832]  x4=[0.134458630057296 8.61341171912092 8.66929297500951;314.159265358979 314.159265358979 314.159265358979;1.04643337073 -0.958079744836906 -2.52599450358573]  x5=1.3417561037125e-06  V1=ones(3,3)  V2=ones(3,3)  I1=ones(3,3)  I2=ones(3,3)  nHarmo=1  Measurements=None  Decoupling=off  VsMag0=0  VrMag0=0  VsAngle0=0  VrAngle0=0  IsMag0=0  IrMag0=0  IsAngle0=0  IrAngle0=0
      settings: SourceProductBaseCode=PS
  Line 48 : spsDistributedParametersLineLib/Distributed Parameters Line  Phases=3  Length=0.3  Frequency=50  Resistance=[0.80718830189013 0.0486237908083191 0.0486712220507153;0.0486237908083191 0.807093436079969 0.0486237934466192;0.0486712220507153 0.0486237934466192 0.80718830189013]  Inductance=[0.00279786707424938 0.00133270803418135 0.00132951476746136;0.00133270803418135 0.00279817608385787 0.00133799988507366;0.00132951476746136 0.00133799988507366 0.00279786707424938]  Capacitance=[7.73340098830622e-09 -1.79942827973291e-09 -1.73218055098733e-09;-1.79942827973291e-09 7.66505189233746e-09 -1.83375898618858e-09;-1.73218055098733e-09 -1.83375898618858e-09 7.749673531177e-09]  x1=[138.663665590896 2395.43262556004 2399.99071699757;314.159265358979 314.159265358979 314.159265358979;1.01908158370176 -0.869022509024962 -2.43812076065424]  x2=[138.663679520059 2395.43277353276 2399.99086550248;314.159265358979 314.159265358979 314.159265358979;1.01908153078096 -0.869022610523503 -2.43812086299802]  x3=[0.120819208169225 6.07804110227068 6.13600421263161;314.159265358979 314.159265358979 314.159265358979;1.01863333217986 -0.869374050491256 -2.43847259950935]  x4=[0.120819208161937 6.07804110234827 6.13600421268307;314.159265358979 314.159265358979 314.159265358979;1.01908153082426 -0.869022610523766 -2.4381208630001]  x5=1.42674452918375e-06  V1=ones(3,3)  V2=ones(3,3)  I1=ones(3,3)  I2=ones(3,3)  nHarmo=1  Measurements=None  Decoupling=off  VsMag0=0  VrMag0=0  VsAngle0=0  VrAngle0=0  IsMag0=0  IrMag0=0  IsAngle0=0  IrAngle0=0
      settings: SourceProductBaseCode=PS
  Line 49 : spsDistributedParametersLineLib/Distributed Parameters Line  Phases=3  Length=0.25999  Frequency=50  Resistance=[0.646656091154803 0.0486237908083191 0.0486712220507153;0.0486237908083191 0.646561225344642 0.0486237934466192;0.0486712220507153 0.0486237934466192 0.646656091154803]  Inductance=[0.00282448912315926 0.00133270803418135 0.00132951476746136;0.00133270803418135 0.00282479813276775 0.00133799988507366;0.00132951476746136 0.00133799988507366 0.00282448912315926]  Capacitance=[7.89543174552926e-09 -1.85986777702161e-09 -1.7901190036642e-09;-1.85986777702161e-09 7.82540023894543e-09 -1.8957321828871e-09;-1.7901190036642e-09 -1.8957321828871e-09 7.91264394645417e-09]  x1=[153.16626200144 2395.45047998511 2399.62815160235;314.159265358979 314.159265358979 314.159265358979;0.937957768708359 -0.864722942987523 -2.43387162571194]  x2=[153.172786670223 2394.9661819526 2399.14537135795;314.159265358979 314.159265358979 314.159265358979;0.937940203212154 -0.864797253653905 -2.43394527873071]  x3=[0.134915355797336 3.7011806589934 3.75702546025825;314.159265358979 314.159265358979 314.159265358979;0.830263083682823 -0.645501007354584 -2.21943739317401]  x4=[0.134453709108485 8.6127815290125 8.66865818123331;314.159265358979 314.159265358979 314.159265358979;1.04561401514548 -0.958587024022194 -2.52650306548558]  x5=1.24573499055177e-06  V1=ones(3,3)  V2=ones(3,3)  I1=ones(3,3)  I2=ones(3,3)  nHarmo=1  Measurements=None  Decoupling=off  VsMag0=0  VrMag0=0  VsAngle0=0  VrAngle0=0  IsMag0=0  IrMag0=0  IsAngle0=0  IrAngle0=0
      settings: SourceProductBaseCode=PS
  Line 5 : spsDistributedParametersLineLib/Distributed Parameters Line  Phases=3  Length=0.3  Frequency=50  Resistance=[0.80718830189013 0.0486237908083191 0.0486712220507153;0.0486237908083191 0.807093436079969 0.0486237934466192;0.0486712220507153 0.0486237934466192 0.80718830189013]  Inductance=[0.00279786707424938 0.00133270803418135 0.00132951476746136;0.00133270803418135 0.00279817608385787 0.00133799988507366;0.00132951476746136 0.00133799988507366 0.00279786707424938]  Capacitance=[7.73340098830622e-09 -1.79942827973291e-09 -1.73218055098733e-09;-1.79942827973291e-09 7.66505189233746e-09 -1.83375898618858e-09;-1.73218055098733e-09 -1.83375898618858e-09 7.749673531177e-09]  x1=[107.500462609785 4217.14236424582 4217.41907050167;314.159265358979 314.159265358979 314.159265358979;0.991157214522269 1.89456284315579 -2.81651600326211]  x2=[107.500473408516 4217.14262475077 4217.41933146413;314.159265358979 314.159265358979 314.159265358979;0.991157161601476 1.89456274165725 -2.8165161056059]  x3=[0.0936663596429122 10.7003488015431 10.7825838657676;314.159265358979 314.159265358979 314.159265358979;0.990708962983361 1.89421130168776 -2.81686784212044]  x4=[0.0936663596347933 10.7003488016239 10.7825838658124;314.159265358979 314.159265358979 314.159265358979;0.991157161673358 1.89456274165892 -2.81651610560492]  x5=1.42674452918375e-06  V1=ones(3,3)  V2=ones(3,3)  I1=ones(3,3)  I2=ones(3,3)  nHarmo=1  Measurements=None  Decoupling=off  VsMag0=0  VrMag0=0  VsAngle0=0  VrAngle0=0  IsMag0=0  IrMag0=0  IsAngle0=0  IrAngle0=0
      settings: SourceProductBaseCode=PS
  Line 50 : spsDistributedParametersLineLib/Distributed Parameters Line  Phases=3  Length=0.02  Frequency=50  Resistance=[0.476003738225748 0.351747138225748 0.351747138225748;0.351747138225748 0.476003738225748 0.351747138225748;0.351747138225748 0.351747138225748 0.476003738225748]  Inductance=[0.000705954362986426 0.000459934243504405 0.000459934243504405;0.000459934243504405 0.000705954362986426 0.000459934243504405;0.000459934243504405 0.000459934243504405 0.000705954362986426]  Capacitance=[5.7561313269996e-07 -1.37543883484145e-07 -1.37543912800485e-07;-1.37543883484145e-07 5.75613027339387e-07 -1.37543875208088e-07;-1.37543912800485e-07 -1.37543875208088e-07 5.75613005057695e-07]  x1=[128.837935945285 2396.08117777163 2400.78105349445;314.159265358979 314.159265358979 314.159265358979;1.07648964815344 -0.782697008854777 -2.35194135410484]  x2=[128.837965700403 2396.07271829091 2400.77259937988;314.159265358979 314.159265358979 314.159265358979;1.07648730573763 -0.782698028208179 -2.35194237792022]  x3=[1.74766444182367 126.100329622406 126.352055682418;314.159265358979 314.159265358979 314.159265358979;1.06999360075573 -0.776252763040746 -2.3455532920447]  x4=[1.7548679328345 131.889848948728 132.144058461658;314.159265358979 314.159265358979 314.159265358979;1.08281808064034 -0.788940769083228 -2.35813182346842]  x5=4.42086352438419e-07  V1=ones(3,3)  V2=ones(3,3)  I1=ones(3,3)  I2=ones(3,3)  nHarmo=1  Measurements=None  Decoupling=off  VsMag0=0  VrMag0=0  VsAngle0=0  VrAngle0=0  IsMag0=0  IrMag0=0  IsAngle0=0  IrAngle0=0
      settings: SourceProductBaseCode=PS
  Line 51 : spsDistributedParametersLineLib/Distributed Parameters Line  Phases=3  Length=1.7101  Frequency=50  Resistance=[0.646656091154803 0.0486237908083191 0.0486712220507153;0.0486237908083191 0.646561225344642 0.0486237934466192;0.0486712220507153 0.0486237934466192 0.646656091154803]  Inductance=[0.00282448912315926 0.00133270803418135 0.00132951476746136;0.00133270803418135 0.00282479813276775 0.00133799988507366;0.00132951476746136 0.00133799988507366 0.00282448912315926]  Capacitance=[7.89543174552926e-09 -1.85986777702161e-09 -1.7901190036642e-09;-1.85986777702161e-09 7.82540023894543e-09 -1.8957321828871e-09;-1.7901190036642e-09 -1.8957321828871e-09 7.91264394645417e-09]  x1=[153.09924130998 2399.69221277407 2403.85856683316;314.159265358979 314.159265358979 314.159265358979;0.935951485708486 -0.865737759602423 -2.43489387046713]  x2=[153.159961726254 2396.08208942732 2400.25795186585;314.159265358979 314.159265358979 314.159265358979;0.935814762725033 -0.866363863862848 -2.43551485577336]  x3=[0.136740627815716 3.30171841742613 3.35618670035136;314.159265358979 314.159265358979 314.159265358979;0.788150701298653 -0.620554709679939 -2.19553284503513]  x4=[0.13377006550012 9.01511131721113 9.07157354208008;314.159265358979 314.159265358979 314.159265358979;1.08431689032525 -0.956567263091218 -2.5245351361288]  x5=8.19389748583632e-06  V1=ones(3,3)  V2=ones(3,3)  I1=ones(3,3)  I2=ones(3,3)  nHarmo=1  Measurements=None  Decoupling=off  VsMag0=0  VrMag0=0  VsAngle0=0  VrAngle0=0  IsMag0=0  IrMag0=0  IsAngle0=0  IrAngle0=0
      settings: SourceProductBaseCode=PS
  Line 52 : spsDistributedParametersLineLib/Distributed Parameters Line  Phases=3  Length=0.02  Frequency=50  Resistance=[0.646656091154803 0.0486237908083191 0.0486712220507153;0.0486237908083191 0.646561225344642 0.0486237934466192;0.0486712220507153 0.0486237934466192 0.646656091154803]  Inductance=[0.00282448912315926 0.00133270803418135 0.00132951476746136;0.00133270803418135 0.00282479813276775 0.00133799988507366;0.00132951476746136 0.00133799988507366 0.00282448912315926]  Capacitance=[7.89543174552926e-09 -1.85986777702161e-09 -1.7901190036642e-09;-1.85986777702161e-09 7.82540023894543e-09 -1.8957321828871e-09;-1.7901190036642e-09 -1.8957321828871e-09 7.91264394645417e-09]  x1=[153.09924130998 2399.69221277407 2403.85856683316;314.159265358979 314.159265358979 314.159265358979;0.938495568812115 -0.863716652666906 -2.43287083958092]  x2=[153.099282437297 2399.68674146234 2403.85309562072;314.159265358979 314.159265358979 314.159265358979;0.938495543536612 -0.863717344169358 -2.43287152282906]  x3=[0.134202384057278 5.75816740188091 5.81507091104032;314.159265358979 314.159265358979 314.159265358979;0.930671501141577 -0.840017809701213 -2.40938206765624]  x4=[0.133523288272987 6.45850807209521 6.51675511551586;314.159265358979 314.159265358979 314.159265358979;0.946329222645216 -0.884868534352955 -2.45385338885618]  x5=9.5829454252223e-08  V1=ones(3,3)  V2=ones(3,3)  I1=ones(3,3)  I2=ones(3,3)  nHarmo=1  Measurements=None  Decoupling=off  VsMag0=0  VrMag0=0  VsAngle0=0  VrAngle0=0  IsMag0=0  IrMag0=0  IsAngle0=0  IrAngle0=0
      settings: SourceProductBaseCode=PS
  Line 53 : spsDistributedParametersLineLib/Distributed Parameters Line  Phases=3  Length=0.02  Frequency=50  Resistance=[0.646656091154803 0.0486237908083191 0.0486712220507153;0.0486237908083191 0.646561225344642 0.0486237934466192;0.0486712220507153 0.0486237934466192 0.646656091154803]  Inductance=[0.00282448912315926 0.00133270803418135 0.00132951476746136;0.00133270803418135 0.00282479813276775 0.00133799988507366;0.00132951476746136 0.00133799988507366 0.00282448912315926]  Capacitance=[7.89543174552926e-09 -1.85986777702161e-09 -1.7901190036642e-09;-1.85986777702161e-09 7.82540023894543e-09 -1.8957321828871e-09;-1.7901190036642e-09 -1.8957321828871e-09 7.91264394645417e-09]  x1=[152.845402136583 2428.55102859105 2432.75491258489;314.159265358979 314.159265358979 314.159265358979;0.9380249265433 -0.854422661952484 -2.42363455212495]  x2=[153.09924130998 2399.69221277407 2403.85856683316;314.159265358979 314.159265358979 314.159265358979;0.938495568812115 -0.863716652666906 -2.43287083958092]  x3=[7.12152813356927 2397.32730990104 2401.55606843061;314.159265358979 314.159265358979 314.159265358979;0.0655314210078194 2.27722348075209 0.708401254992496]  x4=[6.95261605854922 2409.61407315505 2413.95868735521;314.159265358979 314.159265358979 314.159265358979;-3.10553957491107 -0.864342069392163 -2.433165943691]  x5=9.5829454252223e-08  V1=ones(3,3)  V2=ones(3,3)  I1=ones(3,3)  I2=ones(3,3)  nHarmo=1  Measurements=None  Decoupling=off  VsMag0=0  VrMag0=0  VsAngle0=0  VrAngle0=0  IsMag0=0  IrMag0=0  IsAngle0=0  IrAngle0=0
      settings: SourceProductBaseCode=PS
  Line 54 : spsDistributedParametersLineLib/Distributed Parameters Line  Phases=3  Length=1.15  Frequency=50  Resistance=[0.646656091154803 0.0486237908083191 0.0486712220507153;0.0486237908083191 0.646561225344642 0.0486237934466192;0.0486712220507153 0.0486237934466192 0.646656091154803]  Inductance=[0.00282448912315926 0.00133270803418135 0.00132951476746136;0.00133270803418135 0.00282479813276775 0.00133799988507366;0.00132951476746136 0.00133799988507366 0.00282448912315926]  Capacitance=[7.89543174552926e-09 -1.85986777702161e-09 -1.7901190036642e-09;-1.85986777702161e-09 7.82540023894543e-09 -1.8957321828871e-09;-1.7901190036642e-09 -1.8957321828871e-09 7.91264394645417e-09]  x1=[152.845402136583 2428.55102859105 2432.75491258489;314.159265358979 314.159265358979 314.159265358979;0.936323953874759 -0.85577397302114 -2.42498714954605]  x2=[152.848975093667 2428.18756164769 2432.39151737038;314.159265358979 314.159265358979 314.159265358979;0.936319591010207 -0.855819605016045 -2.42503227697767]  x3=[0.133946899687526 5.76959131851211 5.82690614662146;314.159265358979 314.159265358979 314.159265358979;0.923190532110296 -0.829280488395907 -2.39875919754251]  x4=[0.133203087422852 6.57807742836353 6.63694253751984;314.159265358979 314.159265358979 314.159265358979;0.947790106079794 -0.880344671811628 -2.44934880813517]  x5=5.51019361950282e-06  V1=ones(3,3)  V2=ones(3,3)  I1=ones(3,3)  I2=ones(3,3)  nHarmo=1  Measurements=None  Decoupling=off  VsMag0=0  VrMag0=0  VsAngle0=0  VrAngle0=0  IsMag0=0  IrMag0=0  IsAngle0=0  IrAngle0=0
      settings: SourceProductBaseCode=PS
  Line 55 : spsDistributedParametersLineLib/Distributed Parameters Line  Phases=3  Length=0.18999  Frequency=50  Resistance=[0.646656091154803 0.0486237908083191 0.0486712220507153;0.0486237908083191 0.646561225344642 0.0486237934466192;0.0486712220507153 0.0486237934466192 0.646656091154803]  Inductance=[0.00282448912315926 0.00133270803418135 0.00132951476746136;0.00133270803418135 0.00282479813276775 0.00133799988507366;0.00132951476746136 0.00133799988507366 0.00282448912315926]  Capacitance=[7.89543174552926e-09 -1.85986777702161e-09 -1.7901190036642e-09;-1.85986777702161e-09 7.82540023894543e-09 -1.8957321828871e-09;-1.7901190036642e-09 -1.8957321828871e-09 7.91264394645417e-09]  x1=[152.848975093667 2428.18756164769 2432.39151737038;314.159265358979 314.159265358979 314.159265358979;0.937764680188549 -0.854671576574434 -2.42388315569427]  x2=[152.84915030091 2428.16411094676 2432.36807548897;314.159265358979 314.159265358979 314.159265358979;0.937764440073792 -0.854673363856082 -2.4238849112797]  x3=[0.13372997972123 6.03245028077652 6.09038039386303;314.159265358979 314.159265358979 314.159265358979;0.933939568916259 -0.842077019565519 -2.41139605396369]  x4=[0.133529673948785 6.32470442803938 6.38320674009122;314.159265358979 314.159265358979 314.159265358979;0.941309076652875 -0.866907842835432 -2.43602132059502]  x5=9.10331900668992e-07  V1=ones(3,3)  V2=ones(3,3)  I1=ones(3,3)  I2=ones(3,3)  nHarmo=1  Measurements=None  Decoupling=off  VsMag0=0  VrMag0=0  VsAngle0=0  VrAngle0=0  IsMag0=0  IrMag0=0  IsAngle0=0  IrAngle0=0
      settings: SourceProductBaseCode=PS
  Line 56 : spsDistributedParametersLineLib/Distributed Parameters Line  Phases=3  Length=0.34003  Frequency=50  Resistance=[0.646656091154803 0.0486237908083191 0.0486712220507153;0.0486237908083191 0.646561225344642 0.0486237934466192;0.0486712220507153 0.0486237934466192 0.646656091154803]  Inductance=[0.00282448912315926 0.00133270803418135 0.00132951476746136;0.00133270803418135 0.00282479813276775 0.00133799988507366;0.00132951476746136 0.00133799988507366 0.00282448912315926]  Capacitance=[7.89543174552926e-09 -1.85986777702161e-09 -1.7901190036642e-09;-1.85986777702161e-09 7.82540023894543e-09 -1.8957321828871e-09;-1.7901190036642e-09 -1.8957321828871e-09 7.91264394645417e-09]  x1=[152.848975093667 2428.18756164769 2432.39151737038;314.159265358979 314.159265358979 314.159265358979;0.937538827145019 -0.854851001983939 -2.42406275190406]  x2=[152.849619042939 2428.12107168896 2432.32502920852;314.159265358979 314.159265358979 314.159265358979;0.937538246010492 -0.854860778236049 -2.4240724312688]  x3=[0.133894958978265 5.9188518047623 5.97655488584606;314.159265358979 314.159265358979 314.159265358979;0.929944962348396 -0.840414307548342 -2.40976786839232]  x4=[0.133350997798439 6.43634483505827 6.49503279157215;314.159265358979 314.159265358979 314.159265358979;0.944650172330834 -0.868526599384796 -2.43761655910251]  x5=1.62924446646917e-06  V1=ones(3,3)  V2=ones(3,3)  I1=ones(3,3)  I2=ones(3,3)  nHarmo=1  Measurements=None  Decoupling=off  VsMag0=0  VrMag0=0  VsAngle0=0  VrAngle0=0  IsMag0=0  IrMag0=0  IsAngle0=0  IrAngle0=0
      settings: SourceProductBaseCode=PS
  Line 57 : spsDistributedParametersLineLib/Distributed Parameters Line  Phases=3  Length=0.12002  Frequency=50  Resistance=[0.646656091154803 0.0486237908083191 0.0486712220507153;0.0486237908083191 0.646561225344642 0.0486237934466192;0.0486712220507153 0.0486237934466192 0.646656091154803]  Inductance=[0.00282448912315926 0.00133270803418135 0.00132951476746136;0.00133270803418135 0.00282479813276775 0.00133799988507366;0.00132951476746136 0.00133799988507366 0.00282448912315926]  Capacitance=[7.89543174552926e-09 -1.85986777702161e-09 -1.7901190036642e-09;-1.85986777702161e-09 7.82540023894543e-09 -1.8957321828871e-09;-1.7901190036642e-09 -1.8957321828871e-09 7.91264394645417e-09]  x1=[152.849619042939 2428.12107168896 2432.32502920852;314.159265358979 314.159265358979 314.159265358979;0.93786942388377 -0.854597679166832 -2.4238090817479]  x2=[152.849709888031 2428.11030512802 2432.31425516761;314.159265358979 314.159265358979 314.159265358979;0.937869492870454 -0.854600170288236 -2.42381155394605]  x3=[0.133837340850484 6.04479777532788 6.10277890617153;314.159265358979 314.159265358979 314.159265358979;0.935148142715734 -0.851231819168963 -2.42047772787736]  x4=[0.133431581396256 6.31215551407417 6.37062733223471;314.159265358979 314.159265358979 314.159265358979;0.940418106875745 -0.857963905373827 -2.42714343993335]  x5=5.7507255496759e-07  V1=ones(3,3)  V2=ones(3,3)  I1=ones(3,3)  I2=ones(3,3)  nHarmo=1  Measurements=None  Decoupling=off  VsMag0=0  VrMag0=0  VsAngle0=0  VrAngle0=0  IsMag0=0  IrMag0=0  IsAngle0=0  IrAngle0=0
      settings: SourceProductBaseCode=PS
  Line 58 : spsDistributedParametersLineLib/Distributed Parameters Line  Phases=3  Length=0.82  Frequency=50  Resistance=[0.646656091154803 0.0486237908083191 0.0486712220507153;0.0486237908083191 0.646561225344642 0.0486237934466192;0.0486712220507153 0.0486237934466192 0.646656091154803]  Inductance=[0.00282448912315926 0.00133270803418135 0.00132951476746136;0.00133270803418135 0.00282479813276775 0.00133799988507366;0.00132951476746136 0.00133799988507366 0.00282448912315926]  Capacitance=[7.89543174552926e-09 -1.85986777702161e-09 -1.7901190036642e-09;-1.85986777702161e-09 7.82540023894543e-09 -1.8957321828871e-09;-1.7901190036642e-09 -1.8957321828871e-09 7.91264394645417e-09]  x1=[152.849619042939 2428.12107168896 2432.32502920852;314.159265358979 314.159265358979 314.159265358979;0.936815754106314 -0.855434750602087 -2.42464695001588]  x2=[152.850369521621 2428.03246496008 2432.23647127991;314.159265358979 314.159265358979 314.159265358979;0.936814394215875 -0.85544035274603 -2.42465243970577]  x3=[0.133658835968425 6.04877583697535 6.10666871865164;314.159265358979 314.159265358979 314.159265358979;0.932445664752184 -0.844260684110975 -2.41357441272347]  x4=[0.133520601246327 6.29885238973271 6.3572379557983;314.159265358979 314.159265358979 314.159265358979;0.939953869809999 -0.867132087610923 -2.43625091758677]  x5=3.92900762434114e-06  V1=ones(3,3)  V2=ones(3,3)  I1=ones(3,3)  I2=ones(3,3)  nHarmo=1  Measurements=None  Decoupling=off  VsMag0=0  VrMag0=0  VsAngle0=0  VrAngle0=0  IsMag0=0  IrMag0=0  IsAngle0=0  IrAngle0=0
      settings: SourceProductBaseCode=PS
  Line 59 : spsDistributedParametersLineLib/Distributed Parameters Line  Phases=3  Length=1.11  Frequency=50  Resistance=[0.646656091154803 0.0486237908083191 0.0486712220507153;0.0486237908083191 0.646561225344642 0.0486237934466192;0.0486712220507153 0.0486237934466192 0.646656091154803]  Inductance=[0.00282448912315926 0.00133270803418135 0.00132951476746136;0.00133270803418135 0.00282479813276775 0.00133799988507366;0.00132951476746136 0.00133799988507366 0.00282448912315926]  Capacitance=[7.89543174552926e-09 -1.85986777702161e-09 -1.7901190036642e-09;-1.85986777702161e-09 7.82540023894543e-09 -1.8957321828871e-09;-1.7901190036642e-09 -1.8957321828871e-09 7.91264394645417e-09]  x1=[138.811982407814 4221.8723715327 4226.20282401679;314.159265358979 314.159265358979 314.159265358979;0.907577049276692 -0.55814329234818 -2.1290438490954]  x2=[152.845402136583 2428.55102859105 2432.75491258489;314.159265358979 314.159265358979 314.159265358979;0.936384165296655 -0.855726139001011 -2.42493926999132]  x3=[7.11551242037887 2391.69424345402 2395.86766535826;314.159265358979 314.159265358979 314.159265358979;0.0621085046310711 2.27452989814548 0.705705221922652]  x4=[6.95187355949878 2408.09356689983 2412.42093014592;314.159265358979 314.159265358979 314.159265358979;-3.10726229067078 -0.865683444962016 -2.43450847668946]  x5=5.31853471099837e-06  V1=ones(3,3)  V2=ones(3,3)  I1=ones(3,3)  I2=ones(3,3)  nHarmo=1  Measurements=None  Decoupling=off  VsMag0=0  VrMag0=0  VsAngle0=0  VrAngle0=0  IsMag0=0  IrMag0=0  IsAngle0=0  IrAngle0=0
      settings: SourceProductBaseCode=PS
  Line 6 : spsDistributedParametersLineLib/Distributed Parameters Line  Phases=3  Length=0.26  Frequency=50  Resistance=[0.646656091154803 0.0486237908083191 0.0486712220507153;0.0486237908083191 0.646561225344642 0.0486237934466192;0.0486712220507153 0.0486237934466192 0.646656091154803]  Inductance=[0.00282448912315926 0.00133270803418135 0.00132951476746136;0.00133270803418135 0.00282479813276775 0.00133799988507366;0.00132951476746136 0.00133799988507366 0.00282448912315926]  Capacitance=[7.89543174552926e-09 -1.85986777702161e-09 -1.7901190036642e-09;-1.85986777702161e-09 7.82540023894543e-09 -1.8957321828871e-09;-1.7901190036642e-09 -1.8957321828871e-09 7.91264394645417e-09]  x1=[139.624195099916 4217.05366845318 4217.15127755993;314.159265358979 314.159265358979 314.159265358979;0.930888380200773 1.89030920457613 -2.82078799460344]  x2=[139.624205793298 4217.05387228859 4217.15148178833;314.159265358979 314.159265358979 314.159265358979;0.930888347172651 1.89030914307771 -2.82078805662219]  x3=[0.122062872457297 10.7287556234883 10.8113847511496;314.159265358979 314.159265358979 314.159265358979;0.930496989503357 1.88999825269484 -2.82109924272054]  x4=[0.122062872455379 10.7287556234945 10.8113847511017;314.159265358979 314.159265358979 314.159265358979;0.93088834711013 1.89030914307886 -2.82078805662034]  x5=1.2457829052789e-06  V1=ones(3,3)  V2=ones(3,3)  I1=ones(3,3)  I2=ones(3,3)  nHarmo=1  Measurements=None  Decoupling=off  VsMag0=0  VrMag0=0  VsAngle0=0  VrAngle0=0  IsMag0=0  IrMag0=0  IsAngle0=0  IrAngle0=0
      settings: SourceProductBaseCode=PS
  Line 60 : spsDistributedParametersLineLib/Distributed Parameters Line  Phases=3  Length=0.20999  Frequency=50  Resistance=[0.646656091154803 0.0486237908083191 0.0486712220507153;0.0486237908083191 0.646561225344642 0.0486237934466192;0.0486712220507153 0.0486237934466192 0.646656091154803]  Inductance=[0.00282448912315926 0.00133270803418135 0.00132951476746136;0.00133270803418135 0.00282479813276775 0.00133799988507366;0.00132951476746136 0.00133799988507366 0.00282448912315926]  Capacitance=[7.89543174552926e-09 -1.85986777702161e-09 -1.7901190036642e-09;-1.85986777702161e-09 7.82540023894543e-09 -1.8957321828871e-09;-1.7901190036642e-09 -1.8957321828871e-09 7.91264394645417e-09]  x1=[138.811982407814 4221.8723715327 4226.20282401679;314.159265358979 314.159265358979 314.159265358979;0.90893182132219 -0.557067014936763 -2.1279665471441]  x2=[138.817084106079 4221.23093279229 4225.56191292491;314.159265358979 314.159265358979 314.159265358979;0.908950254962818 -0.55715314874449 -2.12805156733641]  x3=[0.132783557725949 6.21549917449588 6.31425875755807;314.159265358979 314.159265358979 314.159265358979;0.838507875954453 -0.445714901965708 -2.01729057607421]  x4=[0.110653683954407 15.3203583611481 15.409111286003;314.159265358979 314.159265358979 314.159265358979;0.993143199130067 -0.602401459998718 -2.17347842257173]  x5=1.00616135492121e-06  V1=ones(3,3)  V2=ones(3,3)  I1=ones(3,3)  I2=ones(3,3)  nHarmo=1  Measurements=None  Decoupling=off  VsMag0=0  VrMag0=0  VsAngle0=0  VrAngle0=0  IsMag0=0  IrMag0=0  IsAngle0=0  IrAngle0=0
      settings: SourceProductBaseCode=PS
  Line 61 : spsDistributedParametersLineLib/Distributed Parameters Line  Phases=3  Length=0.23001  Frequency=50  Resistance=[0.476003738225748 0.351747138225748 0.351747138225748;0.351747138225748 0.476003738225748 0.351747138225748;0.351747138225748 0.351747138225748 0.476003738225748]  Inductance=[0.000705954362986426 0.000459934243504405 0.000459934243504405;0.000459934243504405 0.000705954362986426 0.000459934243504405;0.000459934243504405 0.000459934243504405 0.000705954362986426]  Capacitance=[5.7561313269996e-07 -1.37543883484145e-07 -1.37543912800485e-07;-1.37543883484145e-07 5.75613027339387e-07 -1.37543875208088e-07;-1.37543912800485e-07 -1.37543875208088e-07 5.75613005057695e-07]  x1=[87.1427112342149 4221.68069738207 4226.1840766058;314.159265358979 314.159265358979 314.159265358979;1.07664286887503 -0.476163221331967 -2.04704402890468]  x2=[87.1428682462739 4221.53595808018 4226.03941807389;314.159265358979 314.159265358979 314.159265358979;1.07664457948244 -0.476177018628775 -2.0470577394388]  x3=[1.18218665722574 222.473335799831 222.722331553728;314.159265358979 314.159265358979 314.159265358979;1.07605644805435 -0.473050212841555 -2.04390623984468]  x4=[1.18081627628123 231.590349817894 231.825732737027;314.159265358979 314.159265358979 314.159265358979;1.07563202834402 -0.480105863933685 -2.05101074900107]  x5=5.08421409621804e-06  V1=ones(3,3)  V2=ones(3,3)  I1=ones(3,3)  I2=ones(3,3)  nHarmo=1  Measurements=None  Decoupling=off  VsMag0=0  VrMag0=0  VsAngle0=0  VrAngle0=0  IsMag0=0  IrMag0=0  IsAngle0=0  IrAngle0=0
      settings: SourceProductBaseCode=PS
  Line 62 : spsDistributedParametersLineLib/Distributed Parameters Line  Phases=3  Length=0.24001  Frequency=50  Resistance=[0.646656091154803 0.0486237908083191 0.0486712220507153;0.0486237908083191 0.646561225344642 0.0486237934466192;0.0486712220507153 0.0486237934466192 0.646656091154803]  Inductance=[0.00282448912315926 0.00133270803418135 0.00132951476746136;0.00133270803418135 0.00282479813276775 0.00133799988507366;0.00132951476746136 0.00133799988507366 0.00282448912315926]  Capacitance=[7.89543174552926e-09 -1.85986777702161e-09 -1.7901190036642e-09;-1.85986777702161e-09 7.82540023894543e-09 -1.8957321828871e-09;-1.7901190036642e-09 -1.8957321828871e-09 7.91264394645417e-09]  x1=[135.730671310235 4636.02459239988 4640.07639037921;314.159265358979 314.159265358979 314.159265358979;0.901607896227133 -0.523789973777834 -2.09484848789047]  x2=[138.811982406861 4221.87237170443 4226.20282418839;314.159265358979 314.159265358979 314.159265358979;0.908886632646832 -0.557102914353724 -2.12800248073475]  x3=[7.27700518781536 2397.03669957286 2400.85971480038;314.159265358979 314.159265358979 314.159265358979;0.0673826735687394 2.27563565559091 0.706822741680325]  x4=[7.11863423330422 2418.39270968617 2422.41579505428;314.159265358979 314.159265358979 314.159265358979;-3.09926779975455 -0.862971756603748 -2.43178320255725]  x5=1.1500013657538e-06  V1=ones(3,3)  V2=ones(3,3)  I1=ones(3,3)  I2=ones(3,3)  nHarmo=1  Measurements=None  Decoupling=off  VsMag0=0  VrMag0=0  VsAngle0=0  VrAngle0=0  IsMag0=0  IrMag0=0  IsAngle0=0  IrAngle0=0
      settings: SourceProductBaseCode=PS
  Line 63 : spsDistributedParametersLineLib/Distributed Parameters Line  Phases=3  Length=0.02  Frequency=50  Resistance=[0.646656091154803 0.0486237908083191 0.0486712220507153;0.0486237908083191 0.646561225344642 0.0486237934466192;0.0486712220507153 0.0486237934466192 0.646656091154803]  Inductance=[0.00282448912315926 0.00133270803418135 0.00132951476746136;0.00133270803418135 0.00282479813276775 0.00133799988507366;0.00132951476746136 0.00133799988507366 0.00282448912315926]  Capacitance=[7.89543174552926e-09 -1.85986777702161e-09 -1.7901190036642e-09;-1.85986777702161e-09 7.82540023894543e-09 -1.8957321828871e-09;-1.7901190036642e-09 -1.8957321828871e-09 7.91264394645417e-09]  x1=[135.730671310235 4636.02459239988 4640.07639037921;314.159265358979 314.159265358979 314.159265358979;0.901939074100413 -0.523526874708618 -2.09458513836957]  x2=[135.730691797976 4636.02177491516 4640.07357462993;314.159265358979 314.159265358979 314.159265358979;0.901939125314677 -0.523527091202617 -2.09458535259608]  x3=[0.119060274135447 11.6116416706213 11.7124307083919;314.159265358979 314.159265358979 314.159265358979;0.898326800426349 -0.518148537184028 -2.08925276276208]  x4=[0.118287121089992 11.9844921110612 12.0857061080953;314.159265358979 314.159265358979 314.159265358979;0.90554480553188 -0.528761643088431 -2.09977659954435]  x5=9.5829454252223e-08  V1=ones(3,3)  V2=ones(3,3)  I1=ones(3,3)  I2=ones(3,3)  nHarmo=1  Measurements=None  Decoupling=off  VsMag0=0  VrMag0=0  VsAngle0=0  VrAngle0=0  IsMag0=0  IrMag0=0  IsAngle0=0  IrAngle0=0
      settings: SourceProductBaseCode=PS
  Line 64 : spsDistributedParametersLineLib/Distributed Parameters Line  Phases=3  Length=0.5  Frequency=50  Resistance=[0.646656091154803 0.0486237908083191 0.0486712220507153;0.0486237908083191 0.646561225344642 0.0486237934466192;0.0486712220507153 0.0486237934466192 0.646656091154803]  Inductance=[0.00282448912315926 0.00133270803418135 0.00132951476746136;0.00133270803418135 0.00282479813276775 0.00133799988507366;0.00132951476746136 0.00133799988507366 0.00282448912315926]  Capacitance=[7.89543174552926e-09 -1.85986777702161e-09 -1.7901190036642e-09;-1.85986777702161e-09 7.82540023894543e-09 -1.8957321828871e-09;-1.7901190036642e-09 -1.8957321828871e-09 7.91264394645417e-09]  x1=[129.335761843571 5511.54651336424 5514.91317944969;314.159265358979 314.159265358979 314.159265358979;0.884940412410143 -0.470920764831081 -2.04221151802591]  x2=[135.730671310235 4636.02459239988 4640.07639037921;314.159265358979 314.159265358979 314.159265358979;0.901216537037669 -0.524100882950171 -2.09515969302632]  x3=[7.27463007135705 2394.92881902716 2398.73100145408;314.159265358979 314.159265358979 314.159265358979;0.0662416747288268 2.27472716550736 0.705913218307056]  x4=[7.11973611243131 2418.9889869495 2423.0159096856;314.159265358979 314.159265358979 314.159265358979;-3.09929371336307 -0.862995103591768 -2.43180673498176]  x5=2.39573635630557e-06  V1=ones(3,3)  V2=ones(3,3)  I1=ones(3,3)  I2=ones(3,3)  nHarmo=1  Measurements=None  Decoupling=off  VsMag0=0  VrMag0=0  VsAngle0=0  VrAngle0=0  IsMag0=0  IrMag0=0  IsAngle0=0  IrAngle0=0
      settings: SourceProductBaseCode=PS
  Line 65 : spsDistributedParametersLineLib/Distributed Parameters Line  Phases=3  Length=0.23  Frequency=50  Resistance=[0.646656091154803 0.0486237908083191 0.0486712220507153;0.0486237908083191 0.646561225344642 0.0486237934466192;0.0486712220507153 0.0486237934466192 0.646656091154803]  Inductance=[0.00282448912315926 0.00133270803418135 0.00132951476746136;0.00133270803418135 0.00282479813276775 0.00133799988507366;0.00132951476746136 0.00133799988507366 0.00282448912315926]  Capacitance=[7.89543174552926e-09 -1.85986777702161e-09 -1.7901190036642e-09;-1.85986777702161e-09 7.82540023894543e-09 -1.8957321828871e-09;-1.7901190036642e-09 -1.8957321828871e-09 7.91264394645417e-09]  x1=[126.405282702763 5918.55066438996 5921.57026486324;314.159265358979 314.159265358979 314.159265358979;0.877304322352564 -0.45143492212268 -2.02280200294789]  x2=[129.335761843571 5511.54651336424 5514.91317944969;314.159265358979 314.159265358979 314.159265358979;0.885346839507935 -0.470597885195208 -2.04188833103148]  x3=[7.27706141347983 2395.55499423219 2399.35477416107;314.159265358979 314.159265358979 314.159265358979;0.0663126807962492 2.27479022066137 0.705975410672081]  x4=[7.12555617819242 2422.29778997877 2426.34688703775;314.159265358979 314.159265358979 314.159265358979;-3.0981131339516 -0.862061352597087 -2.43087300928818]  x5=1.10203872390056e-06  V1=ones(3,3)  V2=ones(3,3)  I1=ones(3,3)  I2=ones(3,3)  nHarmo=1  Measurements=None  Decoupling=off  VsMag0=0  VrMag0=0  VsAngle0=0  VrAngle0=0  IsMag0=0  IrMag0=0  IsAngle0=0  IrAngle0=0
      settings: SourceProductBaseCode=PS
  Line 66 : spsDistributedParametersLineLib/Distributed Parameters Line  Phases=3  Length=1.62  Frequency=50  Resistance=[0.80718830189013 0.0486237908083191 0.0486712220507153;0.0486237908083191 0.807093436079969 0.0486237934466192;0.0486712220507153 0.0486237934466192 0.80718830189013]  Inductance=[0.00279786707424938 0.00133270803418135 0.00132951476746136;0.00133270803418135 0.00279817608385787 0.00133799988507366;0.00132951476746136 0.00133799988507366 0.00279786707424938]  Capacitance=[7.73340098830622e-09 -1.79942827973291e-09 -1.73218055098733e-09;-1.79942827973291e-09 7.66505189233746e-09 -1.83375898618858e-09;-1.73218055098733e-09 -1.83375898618858e-09 7.749673531177e-09]  x1=[81.1723542130821 5918.59371218392 5921.81807121156;314.159265358979 314.159265358979 314.159265358979;0.972583435200795 -0.457362072140472 -2.02869710935995]  x2=[81.1728388005386 5918.58456958778 5921.8089647768;314.159265358979 314.159265358979 314.159265358979;0.972583113356315 -0.457365796375539 -2.02870084790833]  x3=[0.0707361931434535 14.975570832488 15.0977766148271;314.159265358979 314.159265358979 314.159265358979;0.969389669854284 -0.45896520038344 -2.03030426946509]  x4=[0.0706071864958558 15.0022836192188 15.1245093419824;314.159265358979 314.159265358979 314.159265358979;0.973359315223305 -0.457663357903362 -2.02899599069431]  x5=7.70442045759223e-06  V1=ones(3,3)  V2=ones(3,3)  I1=ones(3,3)  I2=ones(3,3)  nHarmo=1  Measurements=None  Decoupling=off  VsMag0=0  VrMag0=0  VsAngle0=0  VrAngle0=0  IsMag0=0  IrMag0=0  IsAngle0=0  IrAngle0=0
      settings: SourceProductBaseCode=PS
  Line 67 : spsDistributedParametersLineLib/Distributed Parameters Line  Phases=3  Length=0.54002  Frequency=50  Resistance=[0.646656091154803 0.0486237908083191 0.0486712220507153;0.0486237908083191 0.646561225344642 0.0486237934466192;0.0486712220507153 0.0486237934466192 0.646656091154803]  Inductance=[0.00282448912315926 0.00133270803418135 0.00132951476746136;0.00133270803418135 0.00282479813276775 0.00133799988507366;0.00132951476746136 0.00133799988507366 0.00282448912315926]  Capacitance=[7.89543174552926e-09 -1.85986777702161e-09 -1.7901190036642e-09;-1.85986777702161e-09 7.82540023894543e-09 -1.8957321828871e-09;-1.7901190036642e-09 -1.8957321828871e-09 7.91264394645417e-09]  x1=[119.559199034538 6881.00317137212 6883.15868828472;314.159265358979 314.159265358979 314.159265358979;0.856410135349386 -0.415759628908942 -1.98726055608027]  x2=[126.405282702763 5918.55066438996 5921.57026486325;314.159265358979 314.159265358979 314.159265358979;0.876837653727166 -0.451805659695693 -2.02317309343682]  x3=[7.2740319079829 2393.01553183184 2396.79208679511;314.159265358979 314.159265358979 314.159265358979;0.0650125104415196 2.27378321839613 0.704967503289009]  x4=[7.12615227349861 2422.57049040535 2426.62199548433;314.159265358979 314.159265358979 314.159265358979;-3.09825490619891 -0.862146877636712 -2.4309585579804]  x5=2.58749109426427e-06  V1=ones(3,3)  V2=ones(3,3)  I1=ones(3,3)  I2=ones(3,3)  nHarmo=1  Measurements=None  Decoupling=off  VsMag0=0  VrMag0=0  VsAngle0=0  VrAngle0=0  IsMag0=0  IrMag0=0  IsAngle0=0  IrAngle0=0
      settings: SourceProductBaseCode=PS
  Line 68 : spsDistributedParametersLineLib/Distributed Parameters Line  Phases=3  Length=0.13998  Frequency=50  Resistance=[0.646656091154803 0.0486237908083191 0.0486712220507153;0.0486237908083191 0.646561225344642 0.0486237934466192;0.0486712220507153 0.0486237934466192 0.646656091154803]  Inductance=[0.00282448912315926 0.00133270803418135 0.00132951476746136;0.00133270803418135 0.00282479813276775 0.00133799988507366;0.00132951476746136 0.00133799988507366 0.00282448912315926]  Capacitance=[7.89543174552926e-09 -1.85986777702161e-09 -1.7901190036642e-09;-1.85986777702161e-09 7.82540023894543e-09 -1.8957321828871e-09;-1.7901190036642e-09 -1.8957321828871e-09 7.91264394645417e-09]  x1=[119.559199034538 6881.00317137212 6883.15868828472;314.159265358979 314.159265358979 314.159265358979;0.85701230977976 -0.415281240873627 -1.98678171265342]  x2=[119.560271842797 6880.86483751757 6883.02056153024;314.159265358979 314.159265358979 314.159265358979;0.857015196804966 -0.415285895133238 -1.98678629786587]  x3=[0.107402917723744 16.3108378165329 16.4499624255131;314.159265358979 314.159265358979 314.159265358979;0.826807703602774 -0.380634504805633 -1.95243355484974]  x4=[0.101753356881204 18.7244180581134 18.8651025066007;314.159265358979 314.159265358979 314.159265358979;0.888680890131554 -0.445621508975758 -2.01689227205444]  x5=6.70710350311308e-07  V1=ones(3,3)  V2=ones(3,3)  I1=ones(3,3)  I2=ones(3,3)  nHarmo=1  Measurements=None  Decoupling=off  VsMag0=0  VrMag0=0  VsAngle0=0  VrAngle0=0  IsMag0=0  IrMag0=0  IsAngle0=0  IrAngle0=0
      settings: SourceProductBaseCode=PS
  Line 69 : spsDistributedParametersLineLib/Distributed Parameters Line  Phases=3  Length=0.14997  Frequency=50  Resistance=[0.476003738225748 0.351747138225748 0.351747138225748;0.351747138225748 0.476003738225748 0.351747138225748;0.351747138225748 0.351747138225748 0.476003738225748]  Inductance=[0.000705954362986426 0.000459934243504405 0.000459934243504405;0.000459934243504405 0.000705954362986426 0.000459934243504405;0.000459934243504405 0.000459934243504405 0.000705954362986426]  Capacitance=[5.7561313269996e-07 -1.37543883484145e-07 -1.37543912800485e-07;-1.37543883484145e-07 5.75613027339387e-07 -1.37543875208088e-07;-1.37543912800485e-07 -1.37543875208088e-07 5.75613005057695e-07]  x1=[31.0150041643921 6881.89746987344 6883.96992387273;314.159265358979 314.159265358979 314.159265358979;1.07873404269031 -0.334076781638251 -1.90546678039478]  x2=[31.015020986462 6881.86704374866 6883.9394885852;314.159265358979 314.159265358979 314.159265358979;1.07873279060954 -0.334076965283362 -1.90546696403983]  x3=[0.420913382642869 369.037906318823 369.149011906274;314.159265358979 314.159265358979 314.159265358979;1.07769204481291 -0.332539053596382 -1.90392905213609]  x4=[0.420913327667215 371.450857781071 371.562690000852;314.159265358979 314.159265358979 314.159265358979;1.07873272946186 -0.33622690099121 -1.90761689991395]  x5=3.31498451375949e-06  V1=ones(3,3)  V2=ones(3,3)  I1=ones(3,3)  I2=ones(3,3)  nHarmo=1  Measurements=None  Decoupling=off  VsMag0=0  VrMag0=0  VsAngle0=0  VrAngle0=0  IsMag0=0  IrMag0=0  IsAngle0=0  IrAngle0=0
      settings: SourceProductBaseCode=PS
  Line 7 : spsDistributedParametersLineLib/Distributed Parameters Line  Phases=3  Length=0.02  Frequency=50  Resistance=[0.476003738225748 0.351747138225748 0.351747138225748;0.351747138225748 0.476003738225748 0.351747138225748;0.351747138225748 0.351747138225748 0.476003738225748]  Inductance=[0.000705954362986426 0.000459934243504405 0.000459934243504405;0.000459934243504405 0.000705954362986426 0.000459934243504405;0.000459934243504405 0.000459934243504405 0.000705954362986426]  Capacitance=[5.7561313269996e-07 -1.37543883484145e-07 -1.37543912800485e-07;-1.37543883484145e-07 5.75613027339387e-07 -1.37543875208088e-07;-1.37543912800485e-07 -1.37543875208088e-07 5.75613005057695e-07]  x1=[87.2784175611267 4217.75508115869 4217.45061253617;314.159265358979 314.159265358979 314.159265358979;1.07895571695738 1.8089189637234 -2.90239338526718]  x2=[87.278447466904 4217.75377370592 4217.44930563501;314.159265358979 314.159265358979 314.159265358979;1.07895487993576 1.80891855200136 -2.90239379709784]  x3=[1.18627458046102 226.369783361987 226.353475031708;314.159265358979 314.159265358979 314.159265358979;1.07629866675775 1.80769392581294 -2.90361937456714]  x4=[1.1863980050071 227.755068563417 227.738560249757;314.159265358979 314.159265358979 314.159265358979;1.08147276430837 1.8100531646267 -2.90125823834515]  x5=4.42086352438419e-07  V1=ones(3,3)  V2=ones(3,3)  I1=ones(3,3)  I2=ones(3,3)  nHarmo=1  Measurements=None  Decoupling=off  VsMag0=0  VrMag0=0  VsAngle0=0  VrAngle0=0  IsMag0=0  IrMag0=0  IsAngle0=0  IrAngle0=0
      settings: SourceProductBaseCode=PS
  Line 70 : spsDistributedParametersLineLib/Distributed Parameters Line  Phases=3  Length=0.50001  Frequency=50  Resistance=[0.646656091154803 0.0486237908083191 0.0486712220507153;0.0486237908083191 0.646561225344642 0.0486237934466192;0.0486712220507153 0.0486237934466192 0.646656091154803]  Inductance=[0.00282448912315926 0.00133270803418135 0.00132951476746136;0.00133270803418135 0.00282479813276775 0.00133799988507366;0.00132951476746136 0.00133799988507366 0.00282448912315926]  Capacitance=[7.89543174552926e-09 -1.85986777702161e-09 -1.7901190036642e-09;-1.85986777702161e-09 7.82540023894543e-09 -1.8957321828871e-09;-1.7901190036642e-09 -1.8957321828871e-09 7.91264394645417e-09]  x1=[113.266104751944 7778.70915210443 7780.02288268556;314.159265358979 314.159265358979 314.159265358979;0.835351551078966 -0.390305192655957 -1.96189166640103]  x2=[119.559199034538 6881.00317137212 6883.15868828472;314.159265358979 314.159265358979 314.159265358979;0.856470361824136 -0.415711782930307 -1.98721266455565]  x3=[7.27608163139273 2392.58761114472 2396.3487668321;314.159265358979 314.159265358979 314.159265358979;0.0642864029563718 2.273238557578 0.704420965489837]  x4=[7.13306625587458 2425.956037373 2430.02699232925;314.159265358979 314.159265358979 314.159265358979;-3.09740325199413 -0.861451172553086 -2.43026352549246]  x5=2.3957842710327e-06  V1=ones(3,3)  V2=ones(3,3)  I1=ones(3,3)  I2=ones(3,3)  nHarmo=1  Measurements=None  Decoupling=off  VsMag0=0  VrMag0=0  VsAngle0=0  VrAngle0=0  IsMag0=0  IrMag0=0  IsAngle0=0  IrAngle0=0
      settings: SourceProductBaseCode=PS
  Line 71 : spsDistributedParametersLineLib/Distributed Parameters Line  Phases=3  Length=0.17  Frequency=50  Resistance=[0.646656091154803 0.0486237908083191 0.0486712220507153;0.0486237908083191 0.646561225344642 0.0486237934466192;0.0486712220507153 0.0486237934466192 0.646656091154803]  Inductance=[0.00282448912315926 0.00133270803418135 0.00132951476746136;0.00133270803418135 0.00282479813276775 0.00133799988507366;0.00132951476746136 0.00133799988507366 0.00282448912315926]  Capacitance=[7.89543174552926e-09 -1.85986777702161e-09 -1.7901190036642e-09;-1.85986777702161e-09 7.82540023894543e-09 -1.8957321828871e-09;-1.7901190036642e-09 -1.8957321828871e-09 7.91264394645417e-09]  x1=[113.266104751944 7778.70915210443 7780.02288268556;314.159265358979 314.159265358979 314.159265358979;0.835848310362457 -0.389910550031385 -1.96149664810463]  x2=[113.267146527996 7778.55839554036 7779.87240444853;314.159265358979 314.159265358979 314.159265358979;0.835851565653748 -0.389913628406807 -1.9614996634666]  x3=[0.10141295741044 18.7696529617486 18.9243899075011;314.159265358979 314.159265358979 314.159265358979;0.810644493361241 -0.359381770372467 -1.93122398850942]  x4=[0.0967019205049239 20.830944639107 20.98677658363;314.159265358979 314.159265358979 314.159265358979;0.862021454956603 -0.417613767350157 -1.98898997214697]  x5=8.14550361143895e-07  V1=ones(3,3)  V2=ones(3,3)  I1=ones(3,3)  I2=ones(3,3)  nHarmo=1  Measurements=None  Decoupling=off  VsMag0=0  VrMag0=0  VsAngle0=0  VrAngle0=0  IsMag0=0  IrMag0=0  IsAngle0=0  IrAngle0=0
      settings: SourceProductBaseCode=PS
  Line 72 : spsDistributedParametersLineLib/Distributed Parameters Line  Phases=3  Length=0.27999  Frequency=50  Resistance=[0.646656091154803 0.0486237908083191 0.0486712220507153;0.0486237908083191 0.646561225344642 0.0486237934466192;0.0486712220507153 0.0486237934466192 0.646656091154803]  Inductance=[0.00282448912315926 0.00133270803418135 0.00132951476746136;0.00133270803418135 0.00282479813276775 0.00133799988507366;0.00132951476746136 0.00133799988507366 0.00282448912315926]  Capacitance=[7.89543174552926e-09 -1.85986777702161e-09 -1.7901190036642e-09;-1.85986777702161e-09 7.82540023894543e-09 -1.8957321828871e-09;-1.7901190036642e-09 -1.8957321828871e-09 7.91264394645417e-09]  x1=[109.764460317063 8283.46571988185 8284.29603975146;314.159265358979 314.159265358979 314.159265358979;0.822796799590764 -0.378219931791347 -1.94984354575279]  x2=[113.266104751944 7778.70915210443 7780.02288268556;314.159265358979 314.159265358979 314.159265358979;0.8356827440051 -0.390042081628236 -1.96162830491024]  x3=[7.2787644743974 2393.13843104106 2396.89413544499;314.159265358979 314.159265358979 314.159265358979;0.0641719814660349 2.27315054656478 0.704331679127108]  x4=[7.13938575682117 2429.37591171438 2433.46769088369;314.159265358979 314.159265358979 314.159265358979;-3.0963337905481 -0.86061026766761 -2.42942298965893]  x5=1.341564444804e-06  V1=ones(3,3)  V2=ones(3,3)  I1=ones(3,3)  I2=ones(3,3)  nHarmo=1  Measurements=None  Decoupling=off  VsMag0=0  VrMag0=0  VsAngle0=0  VrAngle0=0  IsMag0=0  IrMag0=0  IsAngle0=0  IrAngle0=0
      settings: SourceProductBaseCode=PS
  Line 73 : spsDistributedParametersLineLib/Distributed Parameters Line  Phases=3  Length=0.01  Frequency=50  Resistance=[0.646656091154803 0.0486237908083191 0.0486712220507153;0.0486237908083191 0.646561225344642 0.0486237934466192;0.0486712220507153 0.0486237934466192 0.646656091154803]  Inductance=[0.00282448912315926 0.00133270803418135 0.00132951476746136;0.00133270803418135 0.00282479813276775 0.00133799988507366;0.00132951476746136 0.00133799988507366 0.00282448912315926]  Capacitance=[7.89543174552926e-09 -1.85986777702161e-09 -1.7901190036642e-09;-1.85986777702161e-09 7.82540023894543e-09 -1.8957321828871e-09;-1.7901190036642e-09 -1.8957321828871e-09 7.91264394645417e-09]  x1=[109.639745003832 8301.51343134655 8302.32636259713;314.159265358979 314.159265358979 314.159265358979;0.822727775288859 -0.377501427092028 -1.94912595694159]  x2=[109.764460317063 8283.46571988185 8284.29603975146;314.159265358979 314.159265358979 314.159265358979;0.823203211635703 -0.377897064113979 -1.94952037072826]  x3=[7.27935859960856 2393.59140665809 2397.3512086657;314.159265358979 314.159265358979 314.159265358979;0.0645637976879979 2.27346096681647 0.704642391228561]  x4=[7.14131877784724 2430.90436787815 2435.01016526255;314.159265358979 314.159265358979 314.159265358979;-3.09550459319695 -0.859953838871519 -2.42876594512851]  x5=4.79147271261115e-08  V1=ones(3,3)  V2=ones(3,3)  I1=ones(3,3)  I2=ones(3,3)  nHarmo=1  Measurements=None  Decoupling=off  VsMag0=0  VrMag0=0  VsAngle0=0  VrAngle0=0  IsMag0=0  IrMag0=0  IsAngle0=0  IrAngle0=0
      settings: SourceProductBaseCode=PS
  Line 74 : spsDistributedParametersLineLib/Distributed Parameters Line  Phases=3  Length=0.04  Frequency=50  Resistance=[0.646656091154803 0.0486237908083191 0.0486712220507153;0.0486237908083191 0.646561225344642 0.0486237934466192;0.0486712220507153 0.0486237934466192 0.646656091154803]  Inductance=[0.00282448912315926 0.00133270803418135 0.00132951476746136;0.00133270803418135 0.00282479813276775 0.00133799988507366;0.00132951476746136 0.00133799988507366 0.00282448912315926]  Capacitance=[7.89543174552926e-09 -1.85986777702161e-09 -1.7901190036642e-09;-1.85986777702161e-09 7.82540023894543e-09 -1.8957321828871e-09;-1.7901190036642e-09 -1.8957321828871e-09 7.91264394645417e-09]  x1=[109.14113274631 8373.71711952788 8374.46041831449;314.159265358979 314.159265358979 314.159265358979;0.820770009966616 -0.375971808717326 -1.94760119501032]  x2=[109.639745003832 8301.51343134655 8302.32636259713;314.159265358979 314.159265358979 314.159265358979;0.822682616722437 -0.377537302607125 -1.94916186660763]  x3=[7.27910018635283 2393.39019046163 2397.14815746775;314.159265358979 314.159265358979 314.159265358979;0.064458616404109 2.27337705088702 0.704558393873211]  x4=[7.14129638982647 2430.88537674287 2434.99099557896;314.159265358979 314.159265358979 314.159265358979;-3.09553459396984 -0.859977863193686 -2.42878999309852]  x5=1.91658908504446e-07  V1=ones(3,3)  V2=ones(3,3)  I1=ones(3,3)  I2=ones(3,3)  nHarmo=1  Measurements=None  Decoupling=off  VsMag0=0  VrMag0=0  VsAngle0=0  VrAngle0=0  IsMag0=0  IrMag0=0  IsAngle0=0  IrAngle0=0
      settings: SourceProductBaseCode=PS
  Line 75 : spsDistributedParametersLineLib/Distributed Parameters Line  Phases=3  Length=0.23  Frequency=50  Resistance=[0.646656091154803 0.0486237908083191 0.0486712220507153;0.0486237908083191 0.646561225344642 0.0486237934466192;0.0486712220507153 0.0486237934466192 0.646656091154803]  Inductance=[0.00282448912315926 0.00133270803418135 0.00132951476746136;0.00133270803418135 0.00282479813276775 0.00133799988507366;0.00132951476746136 0.00133799988507366 0.00282448912315926]  Capacitance=[7.89543174552926e-09 -1.85986777702161e-09 -1.7901190036642e-09;-1.85986777702161e-09 7.82540023894543e-09 -1.8957321828871e-09;-1.7901190036642e-09 -1.8957321828871e-09 7.91264394645417e-09]  x1=[153.199804168261 2393.01687252895 2397.20377423312;314.159265358979 314.159265358979 314.159265358979;0.937902677076418 -0.86506826308985 -2.43421367908923]  x2=[153.203352849777 2392.74528951814 2396.93351438967;314.159265358979 314.159265358979 314.159265358979;0.937890180314666 -0.865113997665535 -2.43425905695974]  x3=[0.133442004034034 4.50538673773574 4.5645554574506;314.159265358979 314.159265358979 314.159265358979;0.867874137093751 -0.761291681657077 -2.33300717987415]  x4=[0.135073841399388 7.70915449254632 7.76363816751589;314.159265358979 314.159265358979 314.159265358979;1.00672728816984 -0.92589945774882 -2.49390483140044]  x5=1.10203872390056e-06  V1=ones(3,3)  V2=ones(3,3)  I1=ones(3,3)  I2=ones(3,3)  nHarmo=1  Measurements=None  Decoupling=off  VsMag0=0  VrMag0=0  VsAngle0=0  VrAngle0=0  IsMag0=0  IrMag0=0  IsAngle0=0  IrAngle0=0
      settings: SourceProductBaseCode=PS
  Line 76 : spsDistributedParametersLineLib/Distributed Parameters Line  Phases=3  Length=1.62  Frequency=50  Resistance=[0.80718830189013 0.0486237908083191 0.0486712220507153;0.0486237908083191 0.807093436079969 0.0486237934466192;0.0486712220507153 0.0486237934466192 0.80718830189013]  Inductance=[0.00279786707424938 0.00133270803418135 0.00132951476746136;0.00133270803418135 0.00279817608385787 0.00133799988507366;0.00132951476746136 0.00133799988507366 0.00279786707424938]  Capacitance=[7.73340098830622e-09 -1.79942827973291e-09 -1.73218055098733e-09;-1.79942827973291e-09 7.66505189233746e-09 -1.83375898618858e-09;-1.73218055098733e-09 -1.83375898618858e-09 7.749673531177e-09]  x1=[138.714768665154 2392.99896519461 2397.56643775608;314.159265358979 314.159265358979 314.159265358979;1.01692681010976 -0.87095018761808 -2.44004645171169]  x2=[138.715281039502 2392.99531591723 2397.56280072424;314.159265358979 314.159265358979 314.159265358979;1.01692519722879 -0.870953847686709 -2.44005012613967]  x3=[0.120783028334913 6.05498880018775 6.11272160538551;314.159265358979 314.159265358979 314.159265358979;1.01424671318479 -0.872541071422181 -2.44164155726835]  x4=[0.12075702081954 6.06562266840903 6.12337511375696;314.159265358979 314.159265358979 314.159265358979;1.01718442381122 -0.871263614363596 -2.44035728442133]  x5=7.70442045759223e-06  V1=ones(3,3)  V2=ones(3,3)  I1=ones(3,3)  I2=ones(3,3)  nHarmo=1  Measurements=None  Decoupling=off  VsMag0=0  VrMag0=0  VsAngle0=0  VrAngle0=0  IsMag0=0  IrMag0=0  IsAngle0=0  IrAngle0=0
      settings: SourceProductBaseCode=PS
  Line 77 : spsDistributedParametersLineLib/Distributed Parameters Line  Phases=3  Length=0.54002  Frequency=50  Resistance=[0.646656091154803 0.0486237908083191 0.0486712220507153;0.0486237908083191 0.646561225344642 0.0486237934466192;0.0486712220507153 0.0486237934466192 0.646656091154803]  Inductance=[0.00282448912315926 0.00133270803418135 0.00132951476746136;0.00133270803418135 0.00282479813276775 0.00133799988507366;0.00132951476746136 0.00133799988507366 0.00282448912315926]  Capacitance=[7.89543174552926e-09 -1.85986777702161e-09 -1.7901190036642e-09;-1.85986777702161e-09 7.82540023894543e-09 -1.8957321828871e-09;-1.7901190036642e-09 -1.8957321828871e-09 7.91264394645417e-09]  x1=[153.191084042464 2393.65310833268 2397.83689042063;314.159265358979 314.159265358979 314.159265358979;0.937466388319211 -0.865329415550619 -2.434476008838]  x2=[153.199804168261 2393.01687252895 2397.20377423312;314.159265358979 314.159265358979 314.159265358979;0.937436008451019 -0.865439000662863 -2.43458476957816]  x3=[0.133453715545682 4.49859681114591 4.55774257615021;314.159265358979 314.159265358979 314.159265358979;0.864105504634325 -0.764414459387264 -2.33613137770004]  x4=[0.135069570142907 7.71193589340212 7.76639801615428;314.159265358979 314.159265358979 314.159265358979;1.00910983162557 -0.924727410486151 -2.49272745743324]  x5=2.58749109426427e-06  V1=ones(3,3)  V2=ones(3,3)  I1=ones(3,3)  I2=ones(3,3)  nHarmo=1  Measurements=None  Decoupling=off  VsMag0=0  VrMag0=0  VsAngle0=0  VrAngle0=0  IsMag0=0  IrMag0=0  IsAngle0=0  IrAngle0=0
      settings: SourceProductBaseCode=PS
  Line 78 : spsDistributedParametersLineLib/Distributed Parameters Line  Phases=3  Length=0.13998  Frequency=50  Resistance=[0.646656091154803 0.0486237908083191 0.0486712220507153;0.0486237908083191 0.646561225344642 0.0486237934466192;0.0486712220507153 0.0486237934466192 0.646656091154803]  Inductance=[0.00282448912315926 0.00133270803418135 0.00132951476746136;0.00133270803418135 0.00282479813276775 0.00133799988507366;0.00132951476746136 0.00133799988507366 0.00282448912315926]  Capacitance=[7.89543174552926e-09 -1.85986777702161e-09 -1.7901190036642e-09;-1.85986777702161e-09 7.82540023894543e-09 -1.8957321828871e-09;-1.7901190036642e-09 -1.8957321828871e-09 7.91264394645417e-09]  x1=[153.191084042464 2393.65310833268 2397.83689042063;314.159265358979 314.159265358979 314.159265358979;0.938068562749585 -0.864851027515305 -2.43399716541115]  x2=[153.191957687247 2393.59623304892 2397.78003380981;314.159265358979 314.159265358979 314.159265358979;0.938067155368319 -0.864855346689866 -2.43400140538829]  x3=[0.134537897727721 5.61626654100678 5.67277686420569;314.159265358979 314.159265358979 314.159265358979;0.912824255101856 -0.819737704924471 -2.3892785071468]  x4=[0.133410626638375 6.57544617131806 6.63385942077401;314.159265358979 314.159265358979 314.159265358979;0.963313202720171 -0.903539178319821 -2.47239310467503]  x5=6.70710350311308e-07  V1=ones(3,3)  V2=ones(3,3)  I1=ones(3,3)  I2=ones(3,3)  nHarmo=1  Measurements=None  Decoupling=off  VsMag0=0  VrMag0=0  VsAngle0=0  VrAngle0=0  IsMag0=0  IrMag0=0  IsAngle0=0  IrAngle0=0
      settings: SourceProductBaseCode=PS
  Line 79 : spsDistributedParametersLineLib/Distributed Parameters Line  Phases=3  Length=0.14997  Frequency=50  Resistance=[0.476003738225748 0.351747138225748 0.351747138225748;0.351747138225748 0.476003738225748 0.351747138225748;0.351747138225748 0.351747138225748 0.476003738225748]  Inductance=[0.000705954362986426 0.000459934243504405 0.000459934243504405;0.000459934243504405 0.000705954362986426 0.000459934243504405;0.000459934243504405 0.000459934243504405 0.000705954362986426]  Capacitance=[5.7561313269996e-07 -1.37543883484145e-07 -1.37543912800485e-07;-1.37543883484145e-07 5.75613027339387e-07 -1.37543875208088e-07;-1.37543912800485e-07 -1.37543875208088e-07 5.75613005057695e-07]  x1=[128.898824975963 2393.59492194717 2398.3027307773;314.159265358979 314.159265358979 314.159265358979;1.07531750871125 -0.783606675757551 -2.35284865992806]  x2=[128.898894878728 2393.58256446688 2398.2903489918;314.159265358979 314.159265358979 314.159265358979;1.07531625642956 -0.7836067086814 -2.35284869285185]  x3=[1.74932226430836 128.295324532066 128.547650437474;314.159265358979 314.159265358979 314.159265358979;1.07427545207528 -0.781626674636839 -2.35086865854913]  x4=[1.74932223747829 129.254443457352 129.508655791373;314.159265358979 314.159265358979 314.159265358979;1.07531625383394 -0.786193926137672 -2.35543591051495]  x5=3.31498451375949e-06  V1=ones(3,3)  V2=ones(3,3)  I1=ones(3,3)  I2=ones(3,3)  nHarmo=1  Measurements=None  Decoupling=off  VsMag0=0  VrMag0=0  VsAngle0=0  VrAngle0=0  IsMag0=0  IrMag0=0  IsAngle0=0  IrAngle0=0
      settings: SourceProductBaseCode=PS
  Line 8 : spsDistributedParametersLineLib/Distributed Parameters Line  Phases=3  Length=1.7101  Frequency=50  Resistance=[0.646656091154803 0.0486237908083191 0.0486712220507153;0.0486237908083191 0.646561225344642 0.0486237934466192;0.0486712220507153 0.0486237934466192 0.646656091154803]  Inductance=[0.00282448912315926 0.00133270803418135 0.00132951476746136;0.00133270803418135 0.00282479813276775 0.00133799988507366;0.00132951476746136 0.00133799988507366 0.00282448912315926]  Capacitance=[7.89543174552926e-09 -1.85986777702161e-09 -1.7901190036642e-09;-1.85986777702161e-09 7.82540023894543e-09 -1.8957321828871e-09;-1.7901190036642e-09 -1.8957321828871e-09 7.91264394645417e-09]  x1=[139.613784628439 4217.52722308047 4217.62642474081;314.159265358979 314.159265358979 314.159265358979;0.928681083305319 1.88877894229394 -2.82232072314351]  x2=[139.623845500539 4217.05071079769 4217.14831403106;314.159265358979 314.159265358979 314.159265358979;0.928709844024047 1.88857704658454 -2.82252179960599]  x3=[0.124384897618616 10.0248441045858 10.1069272565889;314.159265358979 314.159265358979 314.159265358979;0.908250471182206 1.85896217918869 -2.85191616324995]  x4=[0.119605908047925 11.4061523716019 11.488746145149;314.159265358979 314.159265358979 314.159265358979;0.947331114575741 1.91287194182271 -2.7983997697358]  x5=8.19389748583632e-06  V1=ones(3,3)  V2=ones(3,3)  I1=ones(3,3)  I2=ones(3,3)  nHarmo=1  Measurements=None  Decoupling=off  VsMag0=0  VrMag0=0  VsAngle0=0  VrAngle0=0  IsMag0=0  IrMag0=0  IsAngle0=0  IrAngle0=0
      settings: SourceProductBaseCode=PS
  Line 80 : spsDistributedParametersLineLib/Distributed Parameters Line  Phases=3  Length=0.50001  Frequency=50  Resistance=[0.646656091154803 0.0486237908083191 0.0486712220507153;0.0486237908083191 0.646561225344642 0.0486237934466192;0.0486712220507153 0.0486237934466192 0.646656091154803]  Inductance=[0.00282448912315926 0.00133270803418135 0.00132951476746136;0.00133270803418135 0.00282479813276775 0.00133799988507366;0.00132951476746136 0.00133799988507366 0.00282448912315926]  Capacitance=[7.89543174552926e-09 -1.85986777702161e-09 -1.7901190036642e-09;-1.85986777702161e-09 7.82540023894543e-09 -1.8957321828871e-09;-1.7901190036642e-09 -1.8957321828871e-09 7.91264394645417e-09]  x1=[153.179787071803 2394.44438465805 2398.62520742768;314.159265358979 314.159265358979 314.159265358979;0.937560063370167 -0.86516420483674 -2.43431179328235]  x2=[153.191084042464 2393.65310833268 2397.83689042063;314.159265358979 314.159265358979 314.159265358979;0.937526614793962 -0.865281569571985 -2.43442811731338]  x3=[0.134308769627626 4.05944752292542 4.11672068366196;314.159265358979 314.159265358979 314.159265358979;0.838536772348301 -0.691101329962548 -2.26403260454114]  x4=[0.1347999082096 8.21065524430678 8.2658346857388;314.159265358979 314.159265358979 314.159265358979;1.0354366667052 -0.951426581154279 -2.51934255573621]  x5=2.3957842710327e-06  V1=ones(3,3)  V2=ones(3,3)  I1=ones(3,3)  I2=ones(3,3)  nHarmo=1  Measurements=None  Decoupling=off  VsMag0=0  VrMag0=0  VsAngle0=0  VrAngle0=0  IsMag0=0  IrMag0=0  IsAngle0=0  IrAngle0=0
      settings: SourceProductBaseCode=PS
  Line 81 : spsDistributedParametersLineLib/Distributed Parameters Line  Phases=3  Length=0.17  Frequency=50  Resistance=[0.646656091154803 0.0486237908083191 0.0486712220507153;0.0486237908083191 0.646561225344642 0.0486237934466192;0.0486712220507153 0.0486237934466192 0.646656091154803]  Inductance=[0.00282448912315926 0.00133270803418135 0.00132951476746136;0.00133270803418135 0.00282479813276775 0.00133799988507366;0.00132951476746136 0.00133799988507366 0.00282448912315926]  Capacitance=[7.89543174552926e-09 -1.85986777702161e-09 -1.7901190036642e-09;-1.85986777702161e-09 7.82540023894543e-09 -1.8957321828871e-09;-1.7901190036642e-09 -1.8957321828871e-09 7.91264394645417e-09]  x1=[153.179787071803 2394.44438465805 2398.62520742768;314.159265358979 314.159265358979 314.159265358979;0.938056822653658 -0.864769562212167 -2.43391677498595]  x2=[153.180168592331 2394.39633026172 2398.57713742878;314.159265358979 314.159265358979 314.159265358979;0.938056835499628 -0.864778062513915 -2.43392519653895]  x3=[0.134403619281151 5.70388497166561 5.76064593616507;314.159265358979 314.159265358979 314.159265358979;0.929769995808481 -0.846308957720152 -2.4156294054967]  x4=[0.13344441301801 6.48267312935237 6.54090304435067;314.159265358979 314.159265358979 314.159265358979;0.946146404547631 -0.881211297458484 -2.45022174221487]  x5=8.14550361143895e-07  V1=ones(3,3)  V2=ones(3,3)  I1=ones(3,3)  I2=ones(3,3)  nHarmo=1  Measurements=None  Decoupling=off  VsMag0=0  VrMag0=0  VsAngle0=0  VrAngle0=0  IsMag0=0  IrMag0=0  IsAngle0=0  IrAngle0=0
      settings: SourceProductBaseCode=PS
  Line 82 : spsDistributedParametersLineLib/Distributed Parameters Line  Phases=3  Length=0.27999  Frequency=50  Resistance=[0.646656091154803 0.0486237908083191 0.0486712220507153;0.0486237908083191 0.646561225344642 0.0486237934466192;0.0486712220507153 0.0486237934466192 0.646656091154803]  Inductance=[0.00282448912315926 0.00133270803418135 0.00132951476746136;0.00133270803418135 0.00282479813276775 0.00133799988507366;0.00132951476746136 0.00133799988507366 0.00282448912315926]  Capacitance=[7.89543174552926e-09 -1.85986777702161e-09 -1.7901190036642e-09;-1.85986777702161e-09 7.82540023894543e-09 -1.8957321828871e-09;-1.7901190036642e-09 -1.8957321828871e-09 7.91264394645417e-09]  x1=[153.172786670222 2394.9661819526 2399.14537135795;314.159265358979 314.159265358979 314.159265358979;0.937910097501206 -0.86482117066397 -2.43396921850807]  x2=[153.179787071803 2394.44438465805 2398.62520742768;314.159265358979 314.159265358979 314.159265358979;0.937891256296302 -0.864901093809018 -2.43404843179156]  x3=[0.134914348484889 3.70019051936589 3.75602391685423;314.159265358979 314.159265358979 314.159265358979;0.830606036519493 -0.645069411347374 -2.21900836107219]  x4=[0.134452164531428 8.61151964493877 8.66738642157279;314.159265358979 314.159265358979 314.159265358979;1.04514335824643 -0.958918031395612 -2.52683449119169]  x5=1.341564444804e-06  V1=ones(3,3)  V2=ones(3,3)  I1=ones(3,3)  I2=ones(3,3)  nHarmo=1  Measurements=None  Decoupling=off  VsMag0=0  VrMag0=0  VsAngle0=0  VrAngle0=0  IsMag0=0  IrMag0=0  IsAngle0=0  IrAngle0=0
      settings: SourceProductBaseCode=PS
  Line 83 : spsDistributedParametersLineLib/Distributed Parameters Line  Phases=3  Length=0.28003  Frequency=50  Resistance=[0.476003738225748 0.351747138225748 0.351747138225748;0.351747138225748 0.476003738225748 0.351747138225748;0.351747138225748 0.351747138225748 0.476003738225748]  Inductance=[0.000705954362986426 0.000459934243504405 0.000459934243504405;0.000459934243504405 0.000705954362986426 0.000459934243504405;0.000459934243504405 0.000459934243504405 0.000705954362986426]  Capacitance=[5.7561313269996e-07 -1.37543883484145e-07 -1.37543912800485e-07;-1.37543883484145e-07 5.75613027339387e-07 -1.37543875208088e-07;-1.37543912800485e-07 -1.37543875208088e-07 5.75613005057695e-07]  x1=[128.988731614043 2390.89852283072 2395.61456770164;314.159265358979 314.159265358979 314.159265358979;1.07411703804261 -0.784688183838892 -2.35392713295599]  x2=[128.988988155136 2390.90027754143 2395.61632662995;314.159265358979 314.159265358979 314.159265358979;1.07411217914788 -0.784689363520493 -2.35392831350654]  x3=[1.74777193616706 128.546006285443 128.799542125271;314.159265358979 314.159265358979 314.159265358979;1.07206974118538 -0.785901125626002 -2.35514048507717]  x4=[1.74784737876211 128.545993165742 128.799551250949;314.159265358979 314.159265358979 314.159265358979;1.0742126409673 -0.784642252873418 -2.35388079254394]  x5=6.18987206366653e-06  V1=ones(3,3)  V2=ones(3,3)  I1=ones(3,3)  I2=ones(3,3)  nHarmo=1  Measurements=None  Decoupling=off  VsMag0=0  VrMag0=0  VsAngle0=0  VrAngle0=0  IsMag0=0  IrMag0=0  IsAngle0=0  IrAngle0=0
      settings: SourceProductBaseCode=PS
  Line 84 : spsDistributedParametersLineLib/Distributed Parameters Line  Phases=3  Length=0.28003  Frequency=50  Resistance=[0.646656091154803 0.0486237908083191 0.0486712220507153;0.0486237908083191 0.646561225344642 0.0486237934466192;0.0486712220507153 0.0486237934466192 0.646656091154803]  Inductance=[0.00282448912315926 0.00133270803418135 0.00132951476746136;0.00133270803418135 0.00282479813276775 0.00133799988507366;0.00132951476746136 0.00133799988507366 0.00282448912315926]  Capacitance=[7.89543174552926e-09 -1.85986777702161e-09 -1.7901190036642e-09;-1.85986777702161e-09 7.82540023894543e-09 -1.8957321828871e-09;-1.7901190036642e-09 -1.8957321828871e-09 7.91264394645417e-09]  x1=[153.24822380558 2390.90206675235 2395.09401730685;314.159265358979 314.159265358979 314.159265358979;0.937725661236907 -0.865564580720034 -2.43470693132452]  x2=[153.248291456683 2390.90273045124 2395.09468339477;314.159265358979 314.159265358979 314.159265358979;0.937725472430294 -0.865564933915369 -2.43470728747041]  x3=[0.13397253946984 6.08264227402458 6.1400923876857;314.159265358979 314.159265358979 314.159265358979;0.936468935176128 -0.866561087114035 -2.43570431311734]  x4=[0.133971699129418 6.08264241225702 6.14009230736671;314.159265358979 314.159265358979 314.159265358979;0.93856066077048 -0.864903337226573 -2.43404513443033]  x5=1.3417561037125e-06  V1=ones(3,3)  V2=ones(3,3)  I1=ones(3,3)  I2=ones(3,3)  nHarmo=1  Measurements=None  Decoupling=off  VsMag0=0  VrMag0=0  VsAngle0=0  VrAngle0=0  IsMag0=0  IrMag0=0  IsAngle0=0  IrAngle0=0
      settings: SourceProductBaseCode=PS
  Line 85 : spsDistributedParametersLineLib/Distributed Parameters Line  Phases=3  Length=0.3  Frequency=50  Resistance=[0.80718830189013 0.0486237908083191 0.0486712220507153;0.0486237908083191 0.807093436079969 0.0486237934466192;0.0486712220507153 0.0486237934466192 0.80718830189013]  Inductance=[0.00279786707424938 0.00133270803418135 0.00132951476746136;0.00133270803418135 0.00279817608385787 0.00133799988507366;0.00132951476746136 0.00133799988507366 0.00279786707424938]  Capacitance=[7.73340098830622e-09 -1.79942827973291e-09 -1.73218055098733e-09;-1.79942827973291e-09 7.66505189233746e-09 -1.83375898618858e-09;-1.73218055098733e-09 -1.83375898618858e-09 7.749673531177e-09]  x1=[138.779597470192 2390.88475820603 2395.45747387935;314.159265358979 314.159265358979 314.159265358979;1.01872337562551 -0.869840401697536 -2.43893218302202]  x2=[138.779611411 2390.88490589782 2395.45762210377;314.159265358979 314.159265358979 314.159265358979;1.01872332270472 -0.869840503196078 -2.43893228536581]  x3=[0.120920220918138 6.06650158977101 6.12441416827411;314.159265358979 314.159265358979 314.159265358979;1.01827512412316 -0.870191943164006 -2.43928402188626]  x4=[0.120920220908161 6.06650158986448 6.12441416832268;314.159265358979 314.159265358979 314.159265358979;1.01872332272252 -0.869840503196069 -2.438932285359]  x5=1.42674452918375e-06  V1=ones(3,3)  V2=ones(3,3)  I1=ones(3,3)  I2=ones(3,3)  nHarmo=1  Measurements=None  Decoupling=off  VsMag0=0  VrMag0=0  VsAngle0=0  VrAngle0=0  IsMag0=0  IrMag0=0  IsAngle0=0  IrAngle0=0
      settings: SourceProductBaseCode=PS
  Line 86 : spsDistributedParametersLineLib/Distributed Parameters Line  Phases=3  Length=0.26  Frequency=50  Resistance=[0.646656091154803 0.0486237908083191 0.0486712220507153;0.0486237908083191 0.646561225344642 0.0486237934466192;0.0486712220507153 0.0486237934466192 0.646656091154803]  Inductance=[0.00282448912315926 0.00133270803418135 0.00132951476746136;0.00133270803418135 0.00282479813276775 0.00133799988507366;0.00132951476746136 0.00133799988507366 0.00282448912315926]  Capacitance=[7.89543174552926e-09 -1.85986777702161e-09 -1.7901190036642e-09;-1.85986777702161e-09 7.82540023894543e-09 -1.8957321828871e-09;-1.7901190036642e-09 -1.8957321828871e-09 7.91264394645417e-09]  x1=[153.248291456683 2390.90273045124 2395.09468339477;314.159265358979 314.159265358979 314.159265358979;0.937755623299809 -0.865540981029789 -2.43468331178338]  x2=[153.248303193491 2390.90284601786 2395.09479938452;314.159265358979 314.159265358979 314.159265358979;0.937755590271664 -0.86554104252821 -2.43468337380213]  x3=[0.133973389354357 6.08278033221652 6.14023269103427;314.159265358979 314.159265358979 314.159265358979;0.937364232595174 -0.865851932910994 -2.43499455990274]  x4=[0.133973389364928 6.08278033230638 6.14023269105465;314.159265358979 314.159265358979 314.159265358979;0.937755590223216 -0.865541042527493 -2.43468337379792]  x5=1.2457829052789e-06  V1=ones(3,3)  V2=ones(3,3)  I1=ones(3,3)  I2=ones(3,3)  nHarmo=1  Measurements=None  Decoupling=off  VsMag0=0  VrMag0=0  VsAngle0=0  VrAngle0=0  IsMag0=0  IrMag0=0  IsAngle0=0  IrAngle0=0
      settings: SourceProductBaseCode=PS
  Line 87 : spsDistributedParametersLineLib/Distributed Parameters Line  Phases=3  Length=0.02  Frequency=50  Resistance=[0.476003738225748 0.351747138225748 0.351747138225748;0.351747138225748 0.476003738225748 0.351747138225748;0.351747138225748 0.351747138225748 0.476003738225748]  Inductance=[0.000705954362986426 0.000459934243504405 0.000459934243504405;0.000459934243504405 0.000705954362986426 0.000459934243504405;0.000459934243504405 0.000459934243504405 0.000705954362986426]  Capacitance=[5.7561313269996e-07 -1.37543883484145e-07 -1.37543912800485e-07;-1.37543883484145e-07 5.75613027339387e-07 -1.37543875208088e-07;-1.37543912800485e-07 -1.37543875208088e-07 5.75613005057695e-07]  x1=[128.988689725022 2390.89943418794 2395.61548072683;314.159265358979 314.159265358979 314.159265358979;1.07592355402178 -0.783605872165158 -2.35284482121496]  x2=[128.988731614043 2390.89852283072 2395.61456770164;314.159265358979 314.159265358979 314.159265358979;1.07592275817909 -0.783606124154981 -2.35284507335573]  x3=[1.75319317667792 128.340640473335 128.59375466328;314.159265358979 314.159265358979 314.159265358979;1.07339498900875 -0.783728091406804 -2.35296803826634]  x4=[1.75337619729885 129.086839325381 129.341480649578;314.159265358979 314.159265358979 314.159265358979;1.07831216988667 -0.783567598672467 -2.35280555585816]  x5=4.42086352438419e-07  V1=ones(3,3)  V2=ones(3,3)  I1=ones(3,3)  I2=ones(3,3)  nHarmo=1  Measurements=None  Decoupling=off  VsMag0=0  VrMag0=0  VsAngle0=0  VrAngle0=0  IsMag0=0  IrMag0=0  IsAngle0=0  IrAngle0=0
      settings: SourceProductBaseCode=PS
  Line 88 : spsDistributedParametersLineLib/Distributed Parameters Line  Phases=3  Length=1.7101  Frequency=50  Resistance=[0.646656091154803 0.0486237908083191 0.0486712220507153;0.0486237908083191 0.646561225344642 0.0486237934466192;0.0486712220507153 0.0486237934466192 0.646656091154803]  Inductance=[0.00282448912315926 0.00133270803418135 0.00132951476746136;0.00133270803418135 0.00282479813276775 0.00133799988507366;0.00132951476746136 0.00133799988507366 0.00282448912315926]  Capacitance=[7.89543174552926e-09 -1.85986777702161e-09 -1.7901190036642e-09;-1.85986777702161e-09 7.82540023894543e-09 -1.8957321828871e-09;-1.7901190036642e-09 -1.8957321828871e-09 7.91264394645417e-09]  x1=[153.230370640917 2391.26534326387 2395.45779665592;314.159265358979 314.159265358979 314.159265358979;0.93559852231657 -0.867138526370912 -2.43628322946526]  x2=[153.247844667642 2390.90122284938 2395.09317039451;314.159265358979 314.159265358979 314.159265358979;0.935577719873898 -0.86727329926334 -2.43641727613775]  x3=[0.135222305287197 5.7009181481092 5.75754089572169;314.159265358979 314.159265358979 314.159265358979;0.89441393789137 -0.872043968885832 -2.44120179567888]  x4=[0.132736652981181 6.44553193119963 6.50348148511986;314.159265358979 314.159265358979 314.159265358979;0.974934734118997 -0.864854913216756 -2.43398601037912]  x5=8.19389748583632e-06  V1=ones(3,3)  V2=ones(3,3)  I1=ones(3,3)  I2=ones(3,3)  nHarmo=1  Measurements=None  Decoupling=off  VsMag0=0  VrMag0=0  VsAngle0=0  VrAngle0=0  IsMag0=0  IrMag0=0  IsAngle0=0  IrAngle0=0
      settings: SourceProductBaseCode=PS
